simulink model "sliding_car"  (R2017a)
settings: Solver=VariableStepAuto  StartTime=0.0  StopTime=tf  RelTol=1e-3
values from neighbouring files (symbols this model uses):
  R = sys.descrip.syms(end-4)    [load_consts.m]
  sys = kinematic_model(sys)    [load_kin.m]
undefined symbols (not defined in the file or in its folder): a, Cp_1, Cp_2, Fz_1, Fz_2, g, Ic_33, Ii_11, Ii_21, Ii_22, Ii_31, Ii_32, Ii_33, Il_11, Il_21, Il_22, Il_31, Il_32, Il_33, Io_11, Io_21, Io_22, Io_31, Io_32, Io_33, Ir_11, Ir_21, Ir_22, Ir_31, Ir_32, Ir_33, L, Lc, mc, mi, ml, mo, mr, mu_1, mu_2, w, x0
(part 4 of 5)

== matlab function sliding_car/Vehicle/Steering automobile model/Auxiliary matrices/dC_1delta1 ==
  data: x input; qp input; kappa_1 input; kappa_2 input; alpha_1 input; alpha_2 input; dC_1delta output; dkappa_1 input; dkappa_2 input; dalpha_1 input; dalpha_2 input; w parameter; L parameter; R parameter
function dC_1delta = dKinematicMatrix(x, qp, kappa_1, kappa_2, alpha_1, alpha_2, ...
                                      dkappa_1, dkappa_2, dalpha_1, dalpha_2, ... 
                                      w, L, R)
% DCONSTRAINTMATRIX
%    A_1DELTA = DCONSTRAINTMATRIX(L,R,ALPHA_1,ALPHA_2,DELTA_I,DELTA_O,KAPPA_1,KAPPA_2,THETA,W)

%    This function was generated by the Symbolic Math Toolbox version 7.2.
%    16-Oct-2020 14:33:54
    
    x_pos =  x(1);
    y_pos =  x(2);
    theta =  x(3);

    delta_i = x(4);
    delta_o = x(5);

    phi_i = x(6);
    phi_l = x(7);
    phi_o = x(8);
    phi_r = x(9);
    
    p1 = x(10);
    p2 = x(11);
    p3 = x(12);
    
    xp = qp(1);
    yp = qp(2);
    thetap = qp(3);
    deltap_i = qp(4);
    deltap_o = qp(5);
    phip_i = qp(6);
    phip_o = qp(7);
    phip_r = qp(8);
    phip_l = qp(9);
    
    t2 = L.^2;
    t3 = tan(delta_i);
    t4 = t3.^2;
    t5 = tan(alpha_2);
    t6 = t3.*w;
    t7 = L+t6;
    t8 = 1.0./t7.^2;
    t9 = t2.*t4;
    t10 = w.^2;
    t11 = t4.*t10;
    t12 = L.*t3.*w.*2.0;
    t13 = t2+t9+t11+t12;
    t14 = t8.*t13;
    t15 = sqrt(t14);
    t16 = delta_i+theta;
    t17 = cos(t16);
    t18 = delta_o+theta;
    t19 = cos(t18);
    t20 = cos(delta_o);
    t21 = cos(delta_i);
    t22 = sin(delta_o);
    t23 = sin(delta_i);
    t24 = tan(alpha_1);
    t25 = sin(t16);
    t26 = 1.0./t7;
    t27 = L.*t3.*t26;
    t28 = atan(t27);
    t29 = t28+theta;
    t30 = cos(t29);
    t31 = sin(t29);
    t32 = t30.^2;
    t33 = t31.^2;
    t34 = sin(t18);
    t35 = kappa_2.*t2.*t5.*t15.*t19.*t23.*t30.*2.0;
    t36 = kappa_2.*t2.*t5.*t15.*t23.*t30.*t34.*2.0;
    t37 = kappa_2.*t2.*t5.*t15.*t23.*t31.*t34.*2.0;
    t38 = kappa_2.*t3.*t5.*t10.*t15.*t19.*t21.*t30;
    t39 = kappa_2.*t3.*t5.*t10.*t15.*t21.*t30.*t34;
    t40 = L.*kappa_2.*t5.*t15.*t19.*t21.*t30.*w;
    t41 = kappa_2.*t3.*t5.*t10.*t15.*t21.*t31.*t34;
    t42 = L.*kappa_2.*t5.*t15.*t21.*t30.*t34.*w;
    t43 = L.*kappa_2.*t5.*t15.*t21.*t31.*t34.*w;
    t44 = kappa_1.*kappa_2.*t2.*t5.*t15.*t19.*t21.*t24.*t31.*2.0;
    t45 = L.*kappa_2.*t3.*t5.*t15.*t19.*t23.*t30.*w.*2.0;
    t46 = L.*kappa_2.*t3.*t5.*t15.*t23.*t30.*t34.*w.*2.0;
    t47 = L.*kappa_2.*t3.*t5.*t15.*t23.*t31.*t34.*w.*2.0;
    t48 = kappa_1.*kappa_2.*t3.*t5.*t10.*t15.*t19.*t23.*t24.*t30;
    t49 = kappa_1.*kappa_2.*t3.*t5.*t10.*t15.*t23.*t24.*t30.*t34;
    t50 = L.*kappa_1.*kappa_2.*t5.*t15.*t19.*t23.*t24.*t30.*w;
    t51 = kappa_1.*kappa_2.*t3.*t5.*t10.*t15.*t23.*t24.*t31.*t34;
    t52 = L.*kappa_1.*kappa_2.*t5.*t15.*t23.*t24.*t30.*t34.*w;
    t53 = L.*kappa_1.*kappa_2.*t5.*t15.*t23.*t24.*t31.*t34.*w;
    t54 = L.*kappa_1.*kappa_2.*t3.*t5.*t15.*t19.*t21.*t24.*t31.*w.*2.0;
    t55 = t2.*t17.*t31.*2.0;
    t56 = t2.*t15.*t23.*t32.*2.0;
    t57 = t2.*t15.*t23.*t33.*2.0;
    t58 = t3.*t10.*t17.*t30;
    t59 = L.*t17.*t30.*w;
    t60 = t3.*t10.*t25.*t31;
    t61 = L.*t25.*t31.*w;
    t62 = t3.*t10.*t15.*t21.*t32;
    t63 = t3.*t10.*t15.*t21.*t33;
    t64 = L.*t15.*t21.*t32.*w;
    t65 = L.*t15.*t21.*t33.*w;
    t66 = L.*t3.*t17.*t31.*w.*3.0;
    t67 = kappa_1.*t2.*t17.*t24.*t30.*2.0;
    t68 = kappa_1.*t2.*t24.*t25.*t31.*2.0;
    t69 = L.*t3.*t15.*t23.*t32.*w.*2.0;
    t70 = L.*t3.*t15.*t23.*t33.*w.*2.0;
    t71 = kappa_2.*t3.*t5.*t10.*t17.*t19;
    t72 = L.*kappa_2.*t5.*t17.*t19.*w;
    t73 = kappa_2.*t3.*t5.*t10.*t25.*t34;
    t74 = kappa_1.*t2.*t3.*t17.*t24.*t31.*2.0;
    t75 = L.*kappa_2.*t5.*t25.*t34.*w;
    t76 = kappa_1.*t3.*t10.*t24.*t25.*t30;
    t77 = L.*kappa_1.*t24.*t25.*t30.*w;
    t78 = kappa_1.*t3.*t10.*t15.*t23.*t24.*t32;
    t79 = kappa_1.*t3.*t10.*t15.*t23.*t24.*t33;
    t80 = L.*kappa_1.*t15.*t23.*t24.*t32.*w;
    t81 = L.*kappa_1.*t3.*t17.*t24.*t30.*w.*3.0;
    t82 = L.*kappa_1.*t15.*t23.*t24.*t33.*w;
    t83 = kappa_2.*t2.*t5.*t15.*t17.*t20.*t30.*2.0;
    t84 = kappa_2.*t2.*t5.*t15.*t17.*t20.*t31.*2.0;
    t85 = L.*kappa_1.*t3.*t24.*t25.*t31.*w.*3.0;
    t86 = kappa_1.*kappa_2.*t2.*t5.*t17.*t24.*t34.*2.0;
    t87 = kappa_2.*t2.*t5.*t15.*t19.*t23.*t31.*2.0;
    t88 = kappa_2.*t2.*t5.*t15.*t20.*t25.*t31.*2.0;
    t89 = kappa_1.*kappa_2.*t2.*t3.*t5.*t17.*t24.*t34.*2.0;
    t90 = kappa_2.*t3.*t5.*t10.*t15.*t17.*t22.*t30;
    t91 = kappa_2.*t3.*t5.*t10.*t15.*t19.*t21.*t31;
    t92 = kappa_1.*kappa_2.*t3.*t5.*t10.*t19.*t24.*t25;
    t93 = kappa_2.*t3.*t5.*t10.*t15.*t17.*t22.*t31;
    t94 = L.*kappa_2.*t5.*t15.*t17.*t22.*t30.*w;
    t95 = L.*kappa_2.*t5.*t15.*t19.*t21.*t31.*w;
    t96 = kappa_2.*t3.*t5.*t10.*t15.*t22.*t25.*t31;
    t97 = L.*kappa_1.*kappa_2.*t5.*t19.*t24.*t25.*w;
    t98 = L.*kappa_2.*t5.*t15.*t17.*t22.*t31.*w;
    t99 = L.*kappa_2.*t5.*t15.*t22.*t25.*t31.*w;
    t100 = kappa_1.*kappa_2.*t2.*t5.*t15.*t20.*t24.*t25.*t30.*2.0;
    t101 = kappa_1.*kappa_2.*t2.*t5.*t15.*t21.*t24.*t30.*t34.*2.0;
    t102 = kappa_1.*kappa_2.*t2.*t5.*t15.*t20.*t24.*t25.*t31.*2.0;
    t103 = L.*kappa_2.*t3.*t5.*t15.*t17.*t20.*t30.*w.*2.0;
    t104 = L.*kappa_2.*t3.*t5.*t15.*t17.*t20.*t31.*w.*2.0;
    t105 = L.*kappa_1.*kappa_2.*t3.*t5.*t17.*t24.*t34.*w.*3.0;
    t106 = L.*kappa_2.*t3.*t5.*t15.*t19.*t23.*t31.*w.*2.0;
    t107 = L.*kappa_2.*t3.*t5.*t15.*t20.*t25.*t31.*w.*2.0;
    t108 = kappa_1.*kappa_2.*t2.*t5.*t15.*t17.*t20.*t24.*t30.*2.0;
    t109 = kappa_1.*kappa_2.*t3.*t5.*t10.*t15.*t17.*t22.*t24.*t30;
    t110 = kappa_1.*kappa_2.*t3.*t5.*t10.*t15.*t19.*t23.*t24.*t31;
    t111 = kappa_1.*kappa_2.*t3.*t5.*t10.*t15.*t22.*t24.*t25.*t30;
    t112 = L.*kappa_1.*kappa_2.*t5.*t15.*t17.*t22.*t24.*t30.*w;
    t113 = kappa_1.*kappa_2.*t3.*t5.*t10.*t15.*t22.*t24.*t25.*t31;
    t114 = L.*kappa_1.*kappa_2.*t5.*t15.*t19.*t23.*t24.*t31.*w;
    t115 = L.*kappa_1.*kappa_2.*t5.*t15.*t22.*t24.*t25.*t30.*w;
    t116 = L.*kappa_1.*kappa_2.*t5.*t15.*t22.*t24.*t25.*t31.*w;
    t117 = L.*kappa_1.*kappa_2.*t3.*t5.*t15.*t20.*t24.*t25.*t31.*w.*2.0;
    t118 = L.*kappa_1.*kappa_2.*t3.*t5.*t15.*t17.*t20.*t24.*t30.*w.*2.0;
    t119 = L.*kappa_1.*kappa_2.*t3.*t5.*t15.*t20.*t24.*t25.*t30.*w.*2.0;
    t120 = L.*kappa_1.*kappa_2.*t3.*t5.*t15.*t21.*t24.*t30.*t34.*w.*2.0;
    t121 = t5.^2;
    t122 = t121+1.0;
    t149 = t2.*t25.*t30.*2.0;
    t150 = t2.*t3.*t17.*t30.*2.0;
    t151 = t2.*t3.*t25.*t31.*2.0;
    t152 = L.*t3.*t25.*t30.*w.*3.0;
    t153 = kappa_2.*t2.*t5.*t17.*t19.*2.0;
    t154 = kappa_2.*t2.*t5.*t25.*t34.*2.0;
    t155 = kappa_2.*t2.*t3.*t5.*t17.*t19.*2.0;
    t156 = kappa_1.*t2.*t15.*t21.*t24.*t32.*2.0;
    t157 = kappa_2.*t2.*t3.*t5.*t25.*t34.*2.0;
    t158 = kappa_1.*t2.*t15.*t21.*t24.*t33.*2.0;
    t159 = kappa_1.*t2.*t3.*t24.*t25.*t30.*2.0;
    t160 = kappa_1.*t3.*t10.*t17.*t24.*t31;
    t161 = L.*kappa_1.*t17.*t24.*t31.*w;
    t162 = L.*kappa_2.*t3.*t5.*t17.*t19.*w.*3.0;
    t163 = L.*kappa_2.*t3.*t5.*t25.*t34.*w.*3.0;
    t164 = kappa_2.*t2.*t5.*t15.*t20.*t25.*t30.*2.0;
    t165 = kappa_1.*kappa_2.*t2.*t5.*t19.*t24.*t25.*2.0;
    t166 = L.*kappa_1.*t3.*t15.*t21.*t24.*t32.*w.*2.0;
    t167 = L.*kappa_1.*t3.*t15.*t21.*t24.*t33.*w.*2.0;
    t168 = kappa_1.*kappa_2.*t2.*t3.*t5.*t19.*t24.*t25.*2.0;
    t169 = kappa_1.*kappa_2.*t3.*t5.*t10.*t17.*t24.*t34;
    t170 = kappa_2.*t3.*t5.*t10.*t15.*t22.*t25.*t30;
    t171 = L.*kappa_1.*kappa_2.*t5.*t17.*t24.*t34.*w;
    t172 = L.*kappa_2.*t5.*t15.*t22.*t25.*t30.*w;
    t173 = kappa_1.*kappa_2.*t2.*t5.*t15.*t17.*t20.*t24.*t31.*2.0;
    t174 = kappa_1.*kappa_2.*t2.*t5.*t15.*t21.*t24.*t31.*t34.*2.0;
    t175 = L.*kappa_2.*t3.*t5.*t15.*t20.*t25.*t30.*w.*2.0;
    t176 = L.*kappa_1.*kappa_2.*t3.*t5.*t19.*t24.*t25.*w.*3.0;
    t177 = kappa_1.*kappa_2.*t2.*t5.*t15.*t19.*t21.*t24.*t30.*2.0;
    t178 = kappa_1.*kappa_2.*t3.*t5.*t10.*t15.*t17.*t22.*t24.*t31;
    t179 = L.*kappa_1.*kappa_2.*t5.*t15.*t17.*t22.*t24.*t31.*w;
    t180 = L.*kappa_1.*kappa_2.*t3.*t5.*t15.*t21.*t24.*t31.*t34.*w.*2.0;
    t181 = L.*kappa_1.*kappa_2.*t3.*t5.*t15.*t19.*t21.*t24.*t30.*w.*2.0;
    t182 = L.*kappa_1.*kappa_2.*t3.*t5.*t15.*t17.*t20.*t24.*t31.*w.*2.0;
    t123 = t35+t36+t37+t38+t39+t40+t41+t42+t43+t44+t45+t46+t47+t48+t49+t50+t51+t52+t53+t54+t55+t56+t57+t58+t59+t60+t61+t62+t63+t64+t65+t66+t67+t68+t69+t70+t71+t72+t73+t74+t75+t76+t77+t78+t79+t80+t81+t82+t83+t84+t85+t86-t87+t88+t89+t90-t91+t92+t93+t94-t95+t96+t97+t98+t99+t100-t101+t102+t103+t104+t105-t106+t107+t108+t109-t110+t111+t112+t113-t114+t115+t116+t117+t118+t119-t120-t149-t150-t151-t152-t153-t154-t155-t156-t157-t158-t159-t160-t161-t162-t163-t164-t165-t166-t167-t168-t169-t170-t171-t172-t173-t174-t175-t176-t177-t178-t179-t180-t181-t182;
    t124 = L.*R.*t17.*w;
    t125 = R.*t3.*t10.*t17;
    t126 = R.*t2.*t15.*t23.*t30.*2.0;
    t127 = R.*t3.*t10.*t15.*t21.*t30;
    t128 = L.*R.*t15.*t21.*t30.*w;
    t129 = R.*kappa_1.*t3.*t10.*t24.*t25;
    t130 = L.*R.*kappa_1.*t24.*t25.*w;
    t131 = L.*R.*t3.*t15.*t23.*t30.*w.*2.0;
    t132 = R.*kappa_2.*t2.*t5.*t15.*t17.*t20.*2.0;
    t133 = R.*kappa_2.*t2.*t5.*t15.*t23.*t34.*2.0;
    t134 = R.*kappa_2.*t3.*t5.*t10.*t15.*t17.*t22;
    t135 = R.*kappa_2.*t3.*t5.*t10.*t15.*t21.*t34;
    t136 = L.*R.*kappa_2.*t5.*t15.*t17.*t22.*w;
    t137 = L.*R.*kappa_2.*t5.*t15.*t21.*t34.*w;
    t138 = R.*kappa_1.*t3.*t10.*t15.*t23.*t24.*t30;
    t139 = L.*R.*kappa_1.*t15.*t23.*t24.*t30.*w;
    t140 = L.*R.*kappa_2.*t3.*t5.*t15.*t17.*t20.*w.*2.0;
    t141 = L.*R.*kappa_2.*t3.*t5.*t15.*t23.*t34.*w.*2.0;
    t142 = R.*kappa_1.*kappa_2.*t2.*t5.*t15.*t20.*t24.*t25.*2.0;
    t143 = R.*kappa_1.*kappa_2.*t3.*t5.*t10.*t15.*t22.*t24.*t25;
    t144 = R.*kappa_1.*kappa_2.*t3.*t5.*t10.*t15.*t23.*t24.*t34;
    t145 = L.*R.*kappa_1.*kappa_2.*t5.*t15.*t22.*t24.*t25.*w;
    t146 = L.*R.*kappa_1.*kappa_2.*t5.*t15.*t23.*t24.*t34.*w;
    t147 = L.*R.*kappa_1.*kappa_2.*t3.*t5.*t15.*t20.*t24.*t25.*w.*2.0;
    t185 = R.*t2.*t3.*t17.*2.0;
    t186 = R.*kappa_1.*t2.*t3.*t24.*t25.*2.0;
    t187 = R.*kappa_1.*t2.*t15.*t21.*t24.*t30.*2.0;
    t188 = L.*R.*kappa_1.*t3.*t15.*t21.*t24.*t30.*w.*2.0;
    t189 = R.*kappa_1.*kappa_2.*t2.*t5.*t15.*t21.*t24.*t34.*2.0;
    t190 = L.*R.*kappa_1.*kappa_2.*t3.*t5.*t15.*t21.*t24.*t34.*w.*2.0;
    t148 = t124+t125+t126+t127+t128+t129+t130+t131+t132+t133+t134+t135+t136+t137+t138+t139+t140+t141+t142+t143+t144+t145+t146+t147-t185-t186-t187-t188-t189-t190;
    t183 = 1.0./t123.^2;
    t184 = 1.0./t123;
    t191 = t4+1.0;
    t192 = t2.*t3.*t191.*2.0;
    t193 = t3.*t10.*t191.*2.0;
    t194 = L.*t191.*w.*2.0;
    t195 = t192+t193+t194;
    t196 = t8.*t195;
    t197 = 1.0./t7.^3;
    t200 = t13.*t191.*t197.*w.*2.0;
    t198 = t196-t200;
    t199 = 1.0./sqrt(t14);
    t201 = t2.*t4.*t8;
    t202 = t201+1.0;
    t203 = 1.0./t202;
    t204 = L.*t26.*t191;
    t206 = L.*t3.*t8.*t191.*w;
    t205 = t204-t206;
    t207 = kappa_2.*t2.*t5.*t17.*t34.*2.0;
    t208 = kappa_2.*t2.*t3.*t5.*t17.*t34.*2.0;
    t209 = kappa_2.*t3.*t5.*t10.*t19.*t25;
    t210 = L.*kappa_2.*t5.*t19.*t25.*w;
    t211 = L.*kappa_2.*t3.*t5.*t17.*t34.*w.*3.0;
    t212 = kappa_1.*kappa_2.*t2.*t5.*t17.*t19.*t24.*2.0;
    t213 = kappa_1.*kappa_2.*t2.*t5.*t24.*t25.*t34.*2.0;
    t214 = kappa_1.*kappa_2.*t2.*t3.*t5.*t17.*t19.*t24.*2.0;
    t215 = kappa_1.*kappa_2.*t2.*t3.*t5.*t24.*t25.*t34.*2.0;
    t216 = L.*kappa_1.*kappa_2.*t3.*t5.*t17.*t19.*t24.*w.*3.0;
    t217 = L.*kappa_1.*kappa_2.*t3.*t5.*t24.*t25.*t34.*w.*3.0;
    t218 = t24.^2;
    t219 = t218+1.0;
    t220 = R.*t2.*t3.*t25.*2.0;
    t221 = R.*kappa_1.*t3.*t10.*t17.*t24;
    t222 = L.*R.*kappa_1.*t17.*t24.*w;
    t223 = R.*kappa_2.*t2.*t5.*t15.*t19.*t23.*2.0;
    t224 = R.*kappa_2.*t3.*t5.*t10.*t15.*t19.*t21;
    t225 = L.*R.*kappa_2.*t5.*t15.*t19.*t21.*w;
    t226 = L.*R.*kappa_2.*t3.*t5.*t15.*t19.*t23.*w.*2.0;
    t227 = R.*kappa_1.*kappa_2.*t2.*t5.*t15.*t17.*t20.*t24.*2.0;
    t228 = R.*kappa_1.*kappa_2.*t3.*t5.*t10.*t15.*t17.*t22.*t24;
    t229 = R.*kappa_1.*kappa_2.*t3.*t5.*t10.*t15.*t19.*t23.*t24;
    t230 = L.*R.*kappa_1.*kappa_2.*t5.*t15.*t17.*t22.*t24.*w;
    t231 = L.*R.*kappa_1.*kappa_2.*t5.*t15.*t19.*t23.*t24.*w;
    t232 = L.*R.*kappa_1.*kappa_2.*t3.*t5.*t15.*t17.*t20.*t24.*w.*2.0;
    t233 = R.*kappa_1.*t2.*t15.*t21.*t24.*t31.*2.0;
    t234 = L.*R.*kappa_1.*t3.*t15.*t21.*t24.*t31.*w.*2.0;
    t235 = t3.*t5.*t10.*t17.*t19;
    t236 = L.*t5.*t17.*t19.*w;
    t237 = t3.*t5.*t10.*t25.*t34;
    t238 = L.*t5.*t25.*t34.*w;
    t239 = t2.*t5.*t15.*t17.*t20.*t30.*2.0;
    t240 = t2.*t5.*t15.*t17.*t20.*t31.*2.0;
    t241 = t2.*t5.*t15.*t19.*t23.*t30.*2.0;
    t242 = kappa_1.*t2.*t5.*t17.*t24.*t34.*2.0;
    t243 = t2.*t5.*t15.*t20.*t25.*t31.*2.0;
    t244 = t2.*t5.*t15.*t23.*t30.*t34.*2.0;
    t245 = t2.*t5.*t15.*t23.*t31.*t34.*2.0;
    t246 = kappa_1.*t2.*t3.*t5.*t17.*t24.*t34.*2.0;
    t247 = t3.*t5.*t10.*t15.*t19.*t21.*t30;
    t248 = t3.*t5.*t10.*t15.*t17.*t22.*t30;
    t249 = t3.*t5.*t10.*t15.*t21.*t30.*t34;
    t250 = L.*t5.*t15.*t19.*t21.*t30.*w;
    t251 = kappa_1.*t3.*t5.*t10.*t19.*t24.*t25;
    t252 = t3.*t5.*t10.*t15.*t17.*t22.*t31;
    t253 = t3.*t5.*t10.*t15.*t21.*t31.*t34;
    t254 = L.*t5.*t15.*t17.*t22.*t30.*w;
    t255 = L.*t5.*t15.*t21.*t30.*t34.*w;
    t256 = t3.*t5.*t10.*t15.*t22.*t25.*t31;
    t257 = L.*kappa_1.*t5.*t19.*t24.*t25.*w;
    t258 = L.*t5.*t15.*t17.*t22.*t31.*w;
    t259 = L.*t5.*t15.*t21.*t31.*t34.*w;
    t260 = L.*t5.*t15.*t22.*t25.*t31.*w;
    t261 = L.*t3.*t5.*t15.*t17.*t20.*t30.*w.*2.0;
    t262 = L.*t3.*t5.*t15.*t17.*t20.*t31.*w.*2.0;
    t263 = L.*t3.*t5.*t15.*t19.*t23.*t30.*w.*2.0;
    t264 = L.*kappa_1.*t3.*t5.*t17.*t24.*t34.*w.*3.0;
    t265 = L.*t3.*t5.*t15.*t20.*t25.*t31.*w.*2.0;
    t266 = L.*t3.*t5.*t15.*t23.*t30.*t34.*w.*2.0;
    t267 = L.*t3.*t5.*t15.*t23.*t31.*t34.*w.*2.0;
    t268 = kappa_1.*t2.*t5.*t15.*t17.*t20.*t24.*t30.*2.0;
    t269 = kappa_1.*t2.*t5.*t15.*t19.*t21.*t24.*t31.*2.0;
    t270 = kappa_1.*t2.*t5.*t15.*t20.*t24.*t25.*t30.*2.0;
    t271 = kappa_1.*t2.*t5.*t15.*t20.*t24.*t25.*t31.*2.0;
    t272 = kappa_1.*t3.*t5.*t10.*t15.*t17.*t22.*t24.*t30;
    t273 = kappa_1.*t3.*t5.*t10.*t15.*t19.*t23.*t24.*t30;
    t274 = kappa_1.*t3.*t5.*t10.*t15.*t22.*t24.*t25.*t30;
    t275 = kappa_1.*t3.*t5.*t10.*t15.*t23.*t24.*t30.*t34;
    t276 = L.*kappa_1.*t5.*t15.*t17.*t22.*t24.*t30.*w;
    t277 = L.*kappa_1.*t5.*t15.*t19.*t23.*t24.*t30.*w;
    t278 = kappa_1.*t3.*t5.*t10.*t15.*t22.*t24.*t25.*t31;
    t279 = kappa_1.*t3.*t5.*t10.*t15.*t23.*t24.*t31.*t34;
    t280 = L.*kappa_1.*t5.*t15.*t22.*t24.*t25.*t30.*w;
    t281 = L.*kappa_1.*t5.*t15.*t23.*t24.*t30.*t34.*w;
    t282 = L.*kappa_1.*t5.*t15.*t22.*t24.*t25.*t31.*w;
    t283 = L.*kappa_1.*t5.*t15.*t23.*t24.*t31.*t34.*w;
    t284 = L.*kappa_1.*t3.*t5.*t15.*t17.*t20.*t24.*t30.*w.*2.0;
    t285 = L.*kappa_1.*t3.*t5.*t15.*t19.*t21.*t24.*t31.*w.*2.0;
    t286 = L.*kappa_1.*t3.*t5.*t15.*t20.*t24.*t25.*t30.*w.*2.0;
    t287 = L.*kappa_1.*t3.*t5.*t15.*t20.*t24.*t25.*t31.*w.*2.0;
    t641 = t2.*t5.*t17.*t19.*2.0;
    t642 = t2.*t5.*t25.*t34.*2.0;
    t643 = t2.*t3.*t5.*t25.*t34.*2.0;
    t644 = t2.*t3.*t5.*t17.*t19.*2.0;
    t645 = L.*t3.*t5.*t17.*t19.*w.*3.0;
    t646 = L.*t3.*t5.*t25.*t34.*w.*3.0;
    t647 = t2.*t5.*t15.*t20.*t25.*t30.*2.0;
    t648 = kappa_1.*t2.*t5.*t19.*t24.*t25.*2.0;
    t649 = t2.*t5.*t15.*t19.*t23.*t31.*2.0;
    t650 = kappa_1.*t2.*t3.*t5.*t19.*t24.*t25.*2.0;
    t651 = t3.*t5.*t10.*t15.*t19.*t21.*t31;
    t652 = kappa_1.*t3.*t5.*t10.*t17.*t24.*t34;
    t653 = t3.*t5.*t10.*t15.*t22.*t25.*t30;
    t654 = L.*t5.*t15.*t19.*t21.*t31.*w;
    t655 = L.*kappa_1.*t5.*t17.*t24.*t34.*w;
    t656 = L.*t5.*t15.*t22.*t25.*t30.*w;
    t657 = L.*t3.*t5.*t15.*t20.*t25.*t30.*w.*2.0;
    t658 = L.*kappa_1.*t3.*t5.*t19.*t24.*t25.*w.*3.0;
    t659 = L.*t3.*t5.*t15.*t19.*t23.*t31.*w.*2.0;
    t660 = kappa_1.*t2.*t5.*t15.*t19.*t21.*t24.*t30.*2.0;
    t661 = kappa_1.*t2.*t5.*t15.*t17.*t20.*t24.*t31.*2.0;
    t662 = kappa_1.*t2.*t5.*t15.*t21.*t24.*t30.*t34.*2.0;
    t663 = kappa_1.*t2.*t5.*t15.*t21.*t24.*t31.*t34.*2.0;
    t664 = kappa_1.*t3.*t5.*t10.*t15.*t17.*t22.*t24.*t31;
    t665 = kappa_1.*t3.*t5.*t10.*t15.*t19.*t23.*t24.*t31;
    t666 = L.*kappa_1.*t5.*t15.*t17.*t22.*t24.*t31.*w;
    t667 = L.*kappa_1.*t5.*t15.*t19.*t23.*t24.*t31.*w;
    t668 = L.*kappa_1.*t3.*t5.*t15.*t19.*t21.*t24.*t30.*w.*2.0;
    t669 = L.*kappa_1.*t3.*t5.*t15.*t17.*t20.*t24.*t31.*w.*2.0;
    t670 = L.*kappa_1.*t3.*t5.*t15.*t21.*t24.*t30.*t34.*w.*2.0;
    t671 = L.*kappa_1.*t3.*t5.*t15.*t21.*t24.*t31.*t34.*w.*2.0;
    t288 = t235+t236+t237+t238+t239+t240+t241+t242+t243+t244+t245+t246+t247+t248+t249+t250+t251+t252+t253+t254+t255+t256+t257+t258+t259+t260+t261+t262+t263+t264+t265+t266+t267+t268+t269+t270+t271+t272+t273+t274+t275+t276+t277+t278+t279+t280+t281+t282+t283+t284+t285+t286+t287-t641-t642-t643-t644-t645-t646-t647-t648-t649-t650-t651-t652-t653-t654-t655-t656-t657-t658-t659-t660-t661-t662-t663-t664-t665-t666-t667-t668-t669-t670-t671;
    t290 = R.*t3.*t10.*t25;
    t291 = L.*R.*t25.*w;
    t292 = R.*t2.*t15.*t23.*t31.*2.0;
    t293 = R.*kappa_1.*t2.*t3.*t17.*t24.*2.0;
    t294 = R.*t3.*t10.*t15.*t21.*t31;
    t295 = L.*R.*t15.*t21.*t31.*w;
    t296 = L.*R.*t3.*t15.*t23.*t31.*w.*2.0;
    t297 = R.*kappa_2.*t2.*t5.*t15.*t20.*t25.*2.0;
    t298 = R.*kappa_2.*t3.*t5.*t10.*t15.*t22.*t25;
    t299 = L.*R.*kappa_2.*t5.*t15.*t22.*t25.*w;
    t300 = R.*kappa_1.*t3.*t10.*t15.*t23.*t24.*t31;
    t301 = L.*R.*kappa_1.*t15.*t23.*t24.*t31.*w;
    t302 = L.*R.*kappa_2.*t3.*t5.*t15.*t20.*t25.*w.*2.0;
    t303 = R.*kappa_1.*kappa_2.*t2.*t5.*t15.*t19.*t21.*t24.*2.0;
    t304 = L.*R.*kappa_1.*kappa_2.*t3.*t5.*t15.*t19.*t21.*t24.*w.*2.0;
    t289 = t220+t221+t222+t223+t224+t225+t226+t227+t228+t229+t230+t231+t232+t233+t234-t290-t291-t292-t293-t294-t295-t296-t297-t298-t299-t300-t301-t302-t303-t304;
    t305 = kappa_1.*t2.*t17.*t30.*t219.*2.0;
    t306 = kappa_1.*t2.*t25.*t31.*t219.*2.0;
    t307 = kappa_1.*t2.*t3.*t17.*t31.*t219.*2.0;
    t308 = kappa_1.*t3.*t10.*t25.*t30.*t219;
    t309 = L.*kappa_1.*t25.*t30.*t219.*w;
    t310 = kappa_1.*t3.*t10.*t15.*t23.*t32.*t219;
    t311 = kappa_1.*t3.*t10.*t15.*t23.*t33.*t219;
    t312 = L.*kappa_1.*t15.*t23.*t32.*t219.*w;
    t313 = L.*kappa_1.*t3.*t17.*t30.*t219.*w.*3.0;
    t314 = L.*kappa_1.*t15.*t23.*t33.*t219.*w;
    t315 = L.*kappa_1.*t3.*t25.*t31.*t219.*w.*3.0;
    t316 = kappa_1.*kappa_2.*t2.*t5.*t17.*t34.*t219.*2.0;
    t317 = kappa_1.*kappa_2.*t2.*t3.*t5.*t17.*t34.*t219.*2.0;
    t318 = kappa_1.*kappa_2.*t3.*t5.*t10.*t19.*t25.*t219;
    t319 = L.*kappa_1.*kappa_2.*t5.*t19.*t25.*t219.*w;
    t320 = L.*kappa_1.*kappa_2.*t3.*t5.*t17.*t34.*t219.*w.*3.0;
    t321 = kappa_1.*kappa_2.*t2.*t5.*t15.*t17.*t20.*t30.*t219.*2.0;
    t322 = kappa_1.*kappa_2.*t2.*t5.*t15.*t19.*t21.*t31.*t219.*2.0;
    t323 = kappa_1.*kappa_2.*t2.*t5.*t15.*t20.*t25.*t30.*t219.*2.0;
    t324 = kappa_1.*kappa_2.*t2.*t5.*t15.*t20.*t25.*t31.*t219.*2.0;
    t325 = kappa_1.*kappa_2.*t3.*t5.*t10.*t15.*t17.*t22.*t30.*t219;
    t326 = kappa_1.*kappa_2.*t3.*t5.*t10.*t15.*t19.*t23.*t30.*t219;
    t327 = kappa_1.*kappa_2.*t3.*t5.*t10.*t15.*t22.*t25.*t30.*t219;
    t328 = kappa_1.*kappa_2.*t3.*t5.*t10.*t15.*t23.*t30.*t34.*t219;
    t329 = L.*kappa_1.*kappa_2.*t5.*t15.*t17.*t22.*t30.*t219.*w;
    t330 = L.*kappa_1.*kappa_2.*t5.*t15.*t19.*t23.*t30.*t219.*w;
    t331 = kappa_1.*kappa_2.*t3.*t5.*t10.*t15.*t22.*t25.*t31.*t219;
    t332 = kappa_1.*kappa_2.*t3.*t5.*t10.*t15.*t23.*t31.*t34.*t219;
    t333 = L.*kappa_1.*kappa_2.*t5.*t15.*t22.*t25.*t30.*t219.*w;
    t334 = L.*kappa_1.*kappa_2.*t5.*t15.*t23.*t30.*t34.*t219.*w;
    t335 = L.*kappa_1.*kappa_2.*t5.*t15.*t22.*t25.*t31.*t219.*w;
    t336 = L.*kappa_1.*kappa_2.*t5.*t15.*t23.*t31.*t34.*t219.*w;
    t337 = L.*kappa_1.*kappa_2.*t3.*t5.*t15.*t17.*t20.*t30.*t219.*w.*2.0;
    t338 = L.*kappa_1.*kappa_2.*t3.*t5.*t15.*t19.*t21.*t31.*t219.*w.*2.0;
    t339 = L.*kappa_1.*kappa_2.*t3.*t5.*t15.*t20.*t25.*t30.*t219.*w.*2.0;
    t340 = L.*kappa_1.*kappa_2.*t3.*t5.*t15.*t20.*t25.*t31.*t219.*w.*2.0;
    t731 = kappa_1.*t2.*t15.*t21.*t32.*t219.*2.0;
    t732 = kappa_1.*t2.*t15.*t21.*t33.*t219.*2.0;
    t733 = kappa_1.*t2.*t3.*t25.*t30.*t219.*2.0;
    t734 = kappa_1.*t3.*t10.*t17.*t31.*t219;
    t735 = L.*kappa_1.*t17.*t31.*t219.*w;
    t736 = kappa_1.*kappa_2.*t2.*t5.*t19.*t25.*t219.*2.0;
    t737 = L.*kappa_1.*t3.*t15.*t21.*t32.*t219.*w.*2.0;
    t738 = L.*kappa_1.*t3.*t15.*t21.*t33.*t219.*w.*2.0;
    t739 = kappa_1.*kappa_2.*t2.*t3.*t5.*t19.*t25.*t219.*2.0;
    t740 = kappa_1.*kappa_2.*t3.*t5.*t10.*t17.*t34.*t219;
    t741 = L.*kappa_1.*kappa_2.*t5.*t17.*t34.*t219.*w;
    t742 = L.*kappa_1.*kappa_2.*t3.*t5.*t19.*t25.*t219.*w.*3.0;
    t743 = kappa_1.*kappa_2.*t2.*t5.*t15.*t19.*t21.*t30.*t219.*2.0;
    t744 = kappa_1.*kappa_2.*t2.*t5.*t15.*t17.*t20.*t31.*t219.*2.0;
    t745 = kappa_1.*kappa_2.*t2.*t5.*t15.*t21.*t30.*t34.*t219.*2.0;
    t746 = kappa_1.*kappa_2.*t2.*t5.*t15.*t21.*t31.*t34.*t219.*2.0;
    t747 = kappa_1.*kappa_2.*t3.*t5.*t10.*t15.*t17.*t22.*t31.*t219;
    t748 = kappa_1.*kappa_2.*t3.*t5.*t10.*t15.*t19.*t23.*t31.*t219;
    t749 = L.*kappa_1.*kappa_2.*t5.*t15.*t17.*t22.*t31.*t219.*w;
    t750 = L.*kappa_1.*kappa_2.*t5.*t15.*t19.*t23.*t31.*t219.*w;
    t751 = L.*kappa_1.*kappa_2.*t3.*t5.*t15.*t19.*t21.*t30.*t219.*w.*2.0;
    t752 = L.*kappa_1.*kappa_2.*t3.*t5.*t15.*t17.*t20.*t31.*t219.*w.*2.0;
    t753 = L.*kappa_1.*kappa_2.*t3.*t5.*t15.*t21.*t30.*t34.*t219.*w.*2.0;
    t754 = L.*kappa_1.*kappa_2.*t3.*t5.*t15.*t21.*t31.*t34.*t219.*w.*2.0;
    t341 = t305+t306+t307+t308+t309+t310+t311+t312+t313+t314+t315+t316+t317+t318+t319+t320+t321+t322+t323+t324+t325+t326+t327+t328+t329+t330+t331+t332+t333+t334+t335+t336+t337+t338+t339+t340-t731-t732-t733-t734-t735-t736-t737-t738-t739-t740-t741-t742-t743-t744-t745-t746-t747-t748-t749-t750-t751-t752-t753-t754;
    t342 = kappa_2.*t2.*t5.*t19.*t25.*2.0;
    t343 = kappa_2.*t2.*t3.*t5.*t19.*t25.*2.0;
    t344 = kappa_2.*t3.*t5.*t10.*t17.*t34;
    t345 = L.*kappa_2.*t5.*t17.*t34.*w;
    t346 = L.*kappa_2.*t3.*t5.*t19.*t25.*w.*3.0;
    t347 = kappa_2.*t2.*t5.*t15.*t22.*t25.*t30.*2.0;
    t348 = kappa_2.*t3.*t5.*t10.*t15.*t17.*t20.*t30;
    t349 = kappa_1.*kappa_2.*t3.*t5.*t10.*t17.*t19.*t24;
    t350 = kappa_2.*t3.*t5.*t10.*t15.*t17.*t20.*t31;
    t351 = L.*kappa_2.*t5.*t15.*t17.*t20.*t30.*w;
    t352 = kappa_2.*t3.*t5.*t10.*t15.*t20.*t25.*t31;
    t353 = L.*kappa_1.*kappa_2.*t5.*t17.*t19.*t24.*w;
    t354 = L.*kappa_2.*t5.*t15.*t17.*t20.*t31.*w;
    t355 = kappa_1.*kappa_2.*t3.*t5.*t10.*t24.*t25.*t34;
    t356 = L.*kappa_2.*t5.*t15.*t20.*t25.*t31.*w;
    t357 = L.*kappa_1.*kappa_2.*t5.*t24.*t25.*t34.*w;
    t358 = kappa_1.*kappa_2.*t2.*t5.*t15.*t17.*t22.*t24.*t31.*2.0;
    t359 = L.*kappa_2.*t3.*t5.*t15.*t22.*t25.*t30.*w.*2.0;
    t360 = kappa_1.*kappa_2.*t3.*t5.*t10.*t15.*t20.*t24.*t25.*t30;
    t361 = L.*kappa_1.*kappa_2.*t5.*t15.*t17.*t20.*t24.*t30.*w;
    t362 = kappa_1.*kappa_2.*t3.*t5.*t10.*t15.*t20.*t24.*t25.*t31;
    t363 = L.*kappa_1.*kappa_2.*t5.*t15.*t20.*t24.*t25.*t30.*w;
    t364 = L.*kappa_1.*kappa_2.*t5.*t15.*t20.*t24.*t25.*t31.*w;
    t365 = kappa_1.*kappa_2.*t3.*t5.*t10.*t15.*t17.*t20.*t24.*t30;
    t366 = L.*kappa_1.*kappa_2.*t3.*t5.*t15.*t17.*t22.*t24.*t31.*w.*2.0;
    t367 = kappa_2.*t3.*t10.*t17.*t19.*t122;
    t368 = L.*kappa_2.*t17.*t19.*t122.*w;
    t369 = kappa_2.*t3.*t10.*t25.*t34.*t122;
    t370 = L.*kappa_2.*t25.*t34.*t122.*w;
    t371 = kappa_2.*t2.*t15.*t17.*t20.*t30.*t122.*2.0;
    t372 = kappa_2.*t2.*t15.*t17.*t20.*t31.*t122.*2.0;
    t373 = kappa_2.*t2.*t15.*t19.*t23.*t30.*t122.*2.0;
    t374 = kappa_1.*kappa_2.*t2.*t17.*t24.*t34.*t122.*2.0;
    t375 = kappa_2.*t2.*t15.*t20.*t25.*t31.*t122.*2.0;
    t376 = kappa_2.*t2.*t15.*t23.*t30.*t34.*t122.*2.0;
    t377 = kappa_2.*t2.*t15.*t23.*t31.*t34.*t122.*2.0;
    t378 = kappa_1.*kappa_2.*t2.*t3.*t17.*t24.*t34.*t122.*2.0;
    t379 = kappa_2.*t3.*t10.*t15.*t19.*t21.*t30.*t122;
    t380 = kappa_2.*t3.*t10.*t15.*t17.*t22.*t30.*t122;
    t381 = kappa_2.*t3.*t10.*t15.*t21.*t30.*t34.*t122;
    t382 = L.*kappa_2.*t15.*t19.*t21.*t30.*t122.*w;
    t383 = kappa_1.*kappa_2.*t3.*t10.*t19.*t24.*t25.*t122;
    t384 = kappa_2.*t3.*t10.*t15.*t17.*t22.*t31.*t122;
    t385 = kappa_2.*t3.*t10.*t15.*t21.*t31.*t34.*t122;
    t386 = L.*kappa_2.*t15.*t17.*t22.*t30.*t122.*w;
    t387 = L.*kappa_2.*t15.*t21.*t30.*t34.*t122.*w;
    t388 = kappa_2.*t3.*t10.*t15.*t22.*t25.*t31.*t122;
    t389 = L.*kappa_1.*kappa_2.*t19.*t24.*t25.*t122.*w;
    t390 = L.*kappa_2.*t15.*t17.*t22.*t31.*t122.*w;
    t391 = L.*kappa_2.*t15.*t21.*t31.*t34.*t122.*w;
    t392 = L.*kappa_2.*t15.*t22.*t25.*t31.*t122.*w;
    t393 = L.*kappa_2.*t3.*t15.*t17.*t20.*t30.*t122.*w.*2.0;
    t394 = L.*kappa_2.*t3.*t15.*t17.*t20.*t31.*t122.*w.*2.0;
    t395 = L.*kappa_2.*t3.*t15.*t19.*t23.*t30.*t122.*w.*2.0;
    t396 = L.*kappa_1.*kappa_2.*t3.*t17.*t24.*t34.*t122.*w.*3.0;
    t397 = L.*kappa_2.*t3.*t15.*t20.*t25.*t31.*t122.*w.*2.0;
    t398 = L.*kappa_2.*t3.*t15.*t23.*t30.*t34.*t122.*w.*2.0;
    t399 = L.*kappa_2.*t3.*t15.*t23.*t31.*t34.*t122.*w.*2.0;
    t400 = kappa_1.*kappa_2.*t2.*t15.*t17.*t20.*t24.*t30.*t122.*2.0;
    t401 = kappa_1.*kappa_2.*t2.*t15.*t19.*t21.*t24.*t31.*t122.*2.0;
    t402 = kappa_1.*kappa_2.*t2.*t15.*t20.*t24.*t25.*t30.*t122.*2.0;
    t403 = kappa_1.*kappa_2.*t2.*t15.*t20.*t24.*t25.*t31.*t122.*2.0;
    t404 = kappa_1.*kappa_2.*t3.*t10.*t15.*t17.*t22.*t24.*t30.*t122;
    t405 = kappa_1.*kappa_2.*t3.*t10.*t15.*t19.*t23.*t24.*t30.*t122;
    t406 = kappa_1.*kappa_2.*t3.*t10.*t15.*t22.*t24.*t25.*t30.*t122;
    t407 = kappa_1.*kappa_2.*t3.*t10.*t15.*t23.*t24.*t30.*t34.*t122;
    t408 = L.*kappa_1.*kappa_2.*t15.*t17.*t22.*t24.*t30.*t122.*w;
    t409 = L.*kappa_1.*kappa_2.*t15.*t19.*t23.*t24.*t30.*t122.*w;
    t410 = kappa_1.*kappa_2.*t3.*t10.*t15.*t22.*t24.*t25.*t31.*t122;
    t411 = kappa_1.*kappa_2.*t3.*t10.*t15.*t23.*t24.*t31.*t34.*t122;
    t412 = L.*kappa_1.*kappa_2.*t15.*t22.*t24.*t25.*t30.*t122.*w;
    t413 = L.*kappa_1.*kappa_2.*t15.*t23.*t24.*t30.*t34.*t122.*w;
    t414 = L.*kappa_1.*kappa_2.*t15.*t22.*t24.*t25.*t31.*t122.*w;
    t415 = L.*kappa_1.*kappa_2.*t15.*t23.*t24.*t31.*t34.*t122.*w;
    t416 = L.*kappa_1.*kappa_2.*t3.*t15.*t17.*t20.*t24.*t30.*t122.*w.*2.0;
    t417 = L.*kappa_1.*kappa_2.*t3.*t15.*t19.*t21.*t24.*t31.*t122.*w.*2.0;
    t418 = L.*kappa_1.*kappa_2.*t3.*t15.*t20.*t24.*t25.*t30.*t122.*w.*2.0;
    t419 = L.*kappa_1.*kappa_2.*t3.*t15.*t20.*t24.*t25.*t31.*t122.*w.*2.0;
    t700 = kappa_2.*t2.*t17.*t19.*t122.*2.0;
    t701 = kappa_2.*t2.*t25.*t34.*t122.*2.0;
    t702 = kappa_2.*t2.*t3.*t17.*t19.*t122.*2.0;
    t703 = kappa_2.*t2.*t3.*t25.*t34.*t122.*2.0;
    t704 = L.*kappa_2.*t3.*t17.*t19.*t122.*w.*3.0;
    t705 = L.*kappa_2.*t3.*t25.*t34.*t122.*w.*3.0;
    t706 = kappa_2.*t2.*t15.*t20.*t25.*t30.*t122.*2.0;
    t707 = kappa_1.*kappa_2.*t2.*t19.*t24.*t25.*t122.*2.0;
    t708 = kappa_2.*t2.*t15.*t19.*t23.*t31.*t122.*2.0;
    t709 = kappa_1.*kappa_2.*t2.*t3.*t19.*t24.*t25.*t122.*2.0;
    t710 = kappa_2.*t3.*t10.*t15.*t19.*t21.*t31.*t122;
    t711 = kappa_1.*kappa_2.*t3.*t10.*t17.*t24.*t34.*t122;
    t712 = kappa_2.*t3.*t10.*t15.*t22.*t25.*t30.*t122;
    t713 = L.*kappa_2.*t15.*t19.*t21.*t31.*t122.*w;
    t714 = L.*kappa_1.*kappa_2.*t17.*t24.*t34.*t122.*w;
    t715 = L.*kappa_2.*t15.*t22.*t25.*t30.*t122.*w;
    t716 = L.*kappa_2.*t3.*t15.*t20.*t25.*t30.*t122.*w.*2.0;
    t717 = L.*kappa_1.*kappa_2.*t3.*t19.*t24.*t25.*t122.*w.*3.0;
    t718 = L.*kappa_2.*t3.*t15.*t19.*t23.*t31.*t122.*w.*2.0;
    t719 = kappa_1.*kappa_2.*t2.*t15.*t19.*t21.*t24.*t30.*t122.*2.0;
    t720 = kappa_1.*kappa_2.*t2.*t15.*t17.*t20.*t24.*t31.*t122.*2.0;
    t721 = kappa_1.*kappa_2.*t2.*t15.*t21.*t24.*t30.*t34.*t122.*2.0;
    t722 = kappa_1.*kappa_2.*t2.*t15.*t21.*t24.*t31.*t34.*t122.*2.0;
    t723 = kappa_1.*kappa_2.*t3.*t10.*t15.*t17.*t22.*t24.*t31.*t122;
    t724 = kappa_1.*kappa_2.*t3.*t10.*t15.*t19.*t23.*t24.*t31.*t122;
    t725 = L.*kappa_1.*kappa_2.*t15.*t17.*t22.*t24.*t31.*t122.*w;
    t726 = L.*kappa_1.*kappa_2.*t15.*t19.*t23.*t24.*t31.*t122.*w;
    t727 = L.*kappa_1.*kappa_2.*t3.*t15.*t19.*t21.*t24.*t30.*t122.*w.*2.0;
    t728 = L.*kappa_1.*kappa_2.*t3.*t15.*t17.*t20.*t24.*t31.*t122.*w.*2.0;
    t729 = L.*kappa_1.*kappa_2.*t3.*t15.*t21.*t24.*t30.*t34.*t122.*w.*2.0;
    t730 = L.*kappa_1.*kappa_2.*t3.*t15.*t21.*t24.*t31.*t34.*t122.*w.*2.0;
    t420 = t367+t368+t369+t370+t371+t372+t373+t374+t375+t376+t377+t378+t379+t380+t381+t382+t383+t384+t385+t386+t387+t388+t389+t390+t391+t392+t393+t394+t395+t396+t397+t398+t399+t400+t401+t402+t403+t404+t405+t406+t407+t408+t409+t410+t411+t412+t413+t414+t415+t416+t417+t418+t419-t700-t701-t702-t703-t704-t705-t706-t707-t708-t709-t710-t711-t712-t713-t714-t715-t716-t717-t718-t719-t720-t721-t722-t723-t724-t725-t726-t727-t728-t729-t730;
    t421 = t2.*t17.*t24.*t30.*2.0;
    t422 = t2.*t24.*t25.*t31.*2.0;
    t423 = t2.*t3.*t17.*t24.*t31.*2.0;
    t424 = t3.*t10.*t24.*t25.*t30;
    t425 = L.*t24.*t25.*t30.*w;
    t426 = t3.*t10.*t15.*t23.*t24.*t32;
    t427 = t3.*t10.*t15.*t23.*t24.*t33;
    t428 = L.*t15.*t23.*t24.*t32.*w;
    t429 = L.*t3.*t17.*t24.*t30.*w.*3.0;
    t430 = L.*t15.*t23.*t24.*t33.*w;
    t431 = L.*t3.*t24.*t25.*t31.*w.*3.0;
    t432 = kappa_2.*t2.*t5.*t17.*t24.*t34.*2.0;
    t433 = kappa_2.*t2.*t3.*t5.*t17.*t24.*t34.*2.0;
    t434 = kappa_2.*t3.*t5.*t10.*t19.*t24.*t25;
    t435 = L.*kappa_2.*t5.*t19.*t24.*t25.*w;
    t436 = L.*kappa_2.*t3.*t5.*t17.*t24.*t34.*w.*3.0;
    t437 = kappa_2.*t2.*t5.*t15.*t17.*t20.*t24.*t30.*2.0;
    t438 = kappa_2.*t2.*t5.*t15.*t19.*t21.*t24.*t31.*2.0;
    t439 = kappa_2.*t2.*t5.*t15.*t20.*t24.*t25.*t30.*2.0;
    t440 = kappa_2.*t2.*t5.*t15.*t20.*t24.*t25.*t31.*2.0;
    t441 = kappa_2.*t3.*t5.*t10.*t15.*t17.*t22.*t24.*t30;
    t442 = kappa_2.*t3.*t5.*t10.*t15.*t19.*t23.*t24.*t30;
    t443 = kappa_2.*t3.*t5.*t10.*t15.*t22.*t24.*t25.*t30;
    t444 = kappa_2.*t3.*t5.*t10.*t15.*t23.*t24.*t30.*t34;
    t445 = L.*kappa_2.*t5.*t15.*t17.*t22.*t24.*t30.*w;
    t446 = L.*kappa_2.*t5.*t15.*t19.*t23.*t24.*t30.*w;
    t447 = kappa_2.*t3.*t5.*t10.*t15.*t22.*t24.*t25.*t31;
    t448 = kappa_2.*t3.*t5.*t10.*t15.*t23.*t24.*t31.*t34;
    t449 = L.*kappa_2.*t5.*t15.*t22.*t24.*t25.*t30.*w;
    t450 = L.*kappa_2.*t5.*t15.*t23.*t24.*t30.*t34.*w;
    t451 = L.*kappa_2.*t5.*t15.*t22.*t24.*t25.*t31.*w;
    t452 = L.*kappa_2.*t5.*t15.*t23.*t24.*t31.*t34.*w;
    t453 = L.*kappa_2.*t3.*t5.*t15.*t17.*t20.*t24.*t30.*w.*2.0;
    t454 = L.*kappa_2.*t3.*t5.*t15.*t19.*t21.*t24.*t31.*w.*2.0;
    t455 = L.*kappa_2.*t3.*t5.*t15.*t20.*t24.*t25.*t30.*w.*2.0;
    t456 = L.*kappa_2.*t3.*t5.*t15.*t20.*t24.*t25.*t31.*w.*2.0;
    t676 = t2.*t15.*t21.*t24.*t32.*2.0;
    t677 = t2.*t15.*t21.*t24.*t33.*2.0;
    t678 = t2.*t3.*t24.*t25.*t30.*2.0;
    t679 = t3.*t10.*t17.*t24.*t31;
    t680 = L.*t17.*t24.*t31.*w;
    t681 = kappa_2.*t2.*t5.*t19.*t24.*t25.*2.0;
    t682 = L.*t3.*t15.*t21.*t24.*t33.*w.*2.0;
    t683 = kappa_2.*t2.*t3.*t5.*t19.*t24.*t25.*2.0;
    t684 = kappa_2.*t3.*t5.*t10.*t17.*t24.*t34;
    t685 = L.*kappa_2.*t5.*t17.*t24.*t34.*w;
    t686 = L.*t3.*t15.*t21.*t24.*t32.*w.*2.0;
    t687 = L.*kappa_2.*t3.*t5.*t19.*t24.*t25.*w.*3.0;
    t688 = kappa_2.*t2.*t5.*t15.*t19.*t21.*t24.*t30.*2.0;
    t689 = kappa_2.*t2.*t5.*t15.*t17.*t20.*t24.*t31.*2.0;
    t690 = kappa_2.*t2.*t5.*t15.*t21.*t24.*t30.*t34.*2.0;
    t691 = kappa_2.*t2.*t5.*t15.*t21.*t24.*t31.*t34.*2.0;
    t692 = kappa_2.*t3.*t5.*t10.*t15.*t17.*t22.*t24.*t31;
    t693 = kappa_2.*t3.*t5.*t10.*t15.*t19.*t23.*t24.*t31;
    t694 = L.*kappa_2.*t5.*t15.*t17.*t22.*t24.*t31.*w;
    t695 = L.*kappa_2.*t5.*t15.*t19.*t23.*t24.*t31.*w;
    t696 = L.*kappa_2.*t3.*t5.*t15.*t19.*t21.*t24.*t30.*w.*2.0;
    t697 = L.*kappa_2.*t3.*t5.*t15.*t17.*t20.*t24.*t31.*w.*2.0;
    t698 = L.*kappa_2.*t3.*t5.*t15.*t21.*t24.*t30.*t34.*w.*2.0;
    t699 = L.*kappa_2.*t3.*t5.*t15.*t21.*t24.*t31.*t34.*w.*2.0;
    t457 = t421+t422+t423+t424+t425+t426+t427+t428+t429+t430+t431+...
           t432+t433+t434+t435+t436+t437+t438+t439+t440+t441+t442+...
           t443+t444+t445+t446+t447+t448+t449+t450+t451+t452+t453+t454+...
           t455+t456-t676-t677-t678-t679-t680-t681-t682-t683-t684-t685-...
           t686-t687-t688-t689-t690-t691-t692-t693-t694-t695-t696-t697-t698-t699;
    t458 = t2.*t15.*t21.*t32.*2.0;
    t459 = t10.*t17.*t30.*t191;
    t460 = t2.*t15.*t21.*t33.*2.0;
    t461 = t10.*t25.*t31.*t191;
    t462 = t2.*t3.*t25.*t30.*2.0;
    t463 = t3.*t10.*t17.*t31;
    t464 = L.*t17.*t31.*w;
    t465 = t2.*t25.*t31.*t203.*t205.*2.0;
    t466 = t10.*t15.*t21.*t33.*t191;
    t467 = L.*t17.*t31.*t191.*w.*3.0;
    t468 = kappa_1.*t2.*t17.*t24.*t31.*2.0;
    t469 = t2.*t23.*t32.*t198.*t199;
    t470 = t2.*t17.*t30.*t203.*t205.*2.0;
    t471 = t2.*t23.*t33.*t198.*t199;
    t472 = t10.*t15.*t21.*t32.*t191;
    t473 = L.*t15.*t23.*t33.*t191.*w.*2.0;
    t474 = L.*t25.*t30.*t203.*t205.*w;
    t475 = L.*t3.*t15.*t21.*t32.*w.*2.0;
    t476 = L.*t3.*t15.*t21.*t33.*w.*2.0;
    t477 = kappa_2.*t5.*t10.*t17.*t19.*t191;
    t478 = kappa_2.*t5.*t10.*t25.*t34.*t191;
    t479 = kappa_1.*t2.*t17.*t24.*t31.*t191.*2.0;
    t480 = kappa_1.*t2.*t15.*t23.*t24.*t32.*2.0;
    t481 = kappa_1.*t10.*t24.*t25.*t30.*t191;
    t482 = kappa_1.*t2.*t15.*t23.*t24.*t33.*2.0;
    t483 = kappa_1.*t3.*t10.*t17.*t24.*t30;
    t484 = t2.*t3.*t17.*t31.*t203.*t205.*2.0;
    t485 = t3.*t10.*t21.*t32.*t198.*t199.*(1.0./2.0);
    t486 = L.*kappa_1.*t17.*t24.*t30.*w;
    t487 = t3.*t10.*t21.*t33.*t198.*t199.*(1.0./2.0);
    t488 = kappa_1.*t3.*t10.*t24.*t25.*t31;
    t489 = L.*t21.*t32.*t198.*t199.*w.*(1.0./2.0);
    t490 = L.*t21.*t33.*t198.*t199.*w.*(1.0./2.0);
    t491 = L.*kappa_1.*t24.*t25.*t31.*w;
    t492 = t3.*t10.*t25.*t30.*t203.*t205;
    t493 = L.*t15.*t23.*t32.*t191.*w.*2.0;
    t494 = kappa_1.*t2.*t24.*t25.*t30.*t203.*t205.*2.0;
    t495 = kappa_1.*t10.*t15.*t23.*t24.*t32.*t191;
    t496 = kappa_1.*t10.*t15.*t23.*t24.*t33.*t191;
    t497 = L.*kappa_1.*t17.*t24.*t30.*t191.*w.*3.0;
    t498 = kappa_1.*t3.*t10.*t15.*t21.*t24.*t32;
    t499 = L.*kappa_1.*t24.*t25.*t31.*t191.*w.*3.0;
    t500 = kappa_1.*t3.*t10.*t15.*t21.*t24.*t33;
    t501 = L.*kappa_1.*t15.*t21.*t24.*t32.*w;
    t502 = L.*kappa_1.*t15.*t21.*t24.*t33.*w;
    t503 = kappa_2.*t2.*t5.*t15.*t19.*t21.*t30.*2.0;
    t504 = L.*kappa_1.*t3.*t17.*t24.*t31.*w.*3.0;
    t505 = kappa_2.*t2.*t5.*t15.*t21.*t30.*t34.*2.0;
    t506 = L.*t3.*t23.*t32.*t198.*t199.*w;
    t507 = L.*t3.*t17.*t30.*t203.*t205.*w.*3.0;
    t508 = kappa_2.*t2.*t5.*t15.*t21.*t31.*t34.*2.0;
    t509 = L.*t3.*t23.*t33.*t198.*t199.*w;
    t510 = L.*t3.*t25.*t31.*t203.*t205.*w.*3.0;
    t511 = kappa_1.*t2.*t3.*t24.*t25.*t31.*t203.*t205.*2.0;
    t512 = kappa_1.*t3.*t10.*t23.*t24.*t32.*t198.*t199.*(1.0./2.0);
    t513 = kappa_1.*t3.*t10.*t23.*t24.*t33.*t198.*t199.*(1.0./2.0);
    t514 = L.*kappa_1.*t23.*t24.*t32.*t198.*t199.*w.*(1.0./2.0);
    t515 = L.*kappa_1.*t23.*t24.*t33.*t198.*t199.*w.*(1.0./2.0);
    t516 = kappa_2.*t2.*t5.*t17.*t20.*t30.*t198.*t199;
    t517 = kappa_2.*t2.*t5.*t17.*t20.*t31.*t198.*t199;
    t518 = kappa_2.*t2.*t5.*t19.*t23.*t30.*t198.*t199;
    t519 = kappa_2.*t2.*t5.*t20.*t25.*t31.*t198.*t199;
    t520 = kappa_2.*t2.*t5.*t23.*t30.*t34.*t198.*t199;
    t521 = kappa_1.*kappa_2.*t2.*t5.*t17.*t24.*t34.*t191.*2.0;
    t522 = kappa_2.*t5.*t10.*t15.*t19.*t21.*t30.*t191;
    t523 = kappa_2.*t2.*t5.*t23.*t31.*t34.*t198.*t199;
    t524 = L.*kappa_1.*t3.*t15.*t23.*t24.*t32.*w.*2.0;
    t525 = kappa_2.*t5.*t10.*t15.*t17.*t22.*t30.*t191;
    t526 = kappa_2.*t5.*t10.*t15.*t21.*t30.*t34.*t191;
    t527 = L.*kappa_1.*t3.*t15.*t23.*t24.*t33.*w.*2.0;
    t528 = kappa_1.*kappa_2.*t5.*t10.*t19.*t24.*t25.*t191;
    t529 = kappa_2.*t5.*t10.*t15.*t17.*t22.*t31.*t191;
    t530 = kappa_2.*t5.*t10.*t15.*t21.*t31.*t34.*t191;
    t531 = kappa_2.*t5.*t10.*t15.*t22.*t25.*t31.*t191;
    t532 = kappa_2.*t3.*t5.*t10.*t15.*t19.*t23.*t31;
    t533 = L.*kappa_2.*t5.*t15.*t19.*t23.*t31.*w;
    t534 = kappa_1.*t2.*t3.*t17.*t24.*t30.*t203.*t205.*2.0;
    t535 = kappa_1.*kappa_2.*t2.*t5.*t15.*t19.*t23.*t24.*t30.*2.0;
    t536 = kappa_1.*kappa_2.*t2.*t5.*t15.*t23.*t24.*t30.*t34.*2.0;
    t537 = kappa_2.*t2.*t5.*t15.*t17.*t20.*t30.*t203.*t205.*2.0;
    t538 = L.*kappa_1.*t3.*t24.*t25.*t30.*t203.*t205.*w.*3.0;
    t539 = kappa_1.*kappa_2.*t2.*t5.*t15.*t23.*t24.*t31.*t34.*2.0;
    t540 = kappa_2.*t2.*t5.*t15.*t20.*t25.*t30.*t203.*t205.*2.0;
    t541 = kappa_2.*t2.*t5.*t15.*t20.*t25.*t31.*t203.*t205.*2.0;
    t542 = kappa_2.*t2.*t5.*t15.*t23.*t30.*t34.*t203.*t205.*2.0;
    t543 = kappa_2.*t3.*t5.*t10.*t19.*t21.*t30.*t198.*t199.*(1.0./2.0);
    t544 = kappa_2.*t3.*t5.*t10.*t17.*t22.*t30.*t198.*t199.*(1.0./2.0);
    t545 = kappa_2.*t3.*t5.*t10.*t21.*t30.*t34.*t198.*t199.*(1.0./2.0);
    t546 = L.*kappa_2.*t5.*t19.*t21.*t30.*t198.*t199.*w.*(1.0./2.0);
    t547 = L.*kappa_2.*t5.*t15.*t17.*t20.*t30.*t191.*w.*2.0;
    t548 = kappa_2.*t3.*t5.*t10.*t17.*t22.*t31.*t198.*t199.*(1.0./2.0);
    t549 = kappa_2.*t3.*t5.*t10.*t21.*t31.*t34.*t198.*t199.*(1.0./2.0);
    t550 = L.*kappa_2.*t5.*t17.*t22.*t30.*t198.*t199.*w.*(1.0./2.0);
    t551 = L.*kappa_2.*t5.*t21.*t30.*t34.*t198.*t199.*w.*(1.0./2.0);
    t552 = L.*kappa_2.*t5.*t15.*t17.*t20.*t31.*t191.*w.*2.0;
    t553 = L.*kappa_2.*t5.*t15.*t19.*t23.*t30.*t191.*w.*2.0;
    t554 = kappa_2.*t3.*t5.*t10.*t22.*t25.*t31.*t198.*t199.*(1.0./2.0);
    t555 = L.*kappa_2.*t5.*t17.*t22.*t31.*t198.*t199.*w.*(1.0./2.0);
    t556 = L.*kappa_2.*t5.*t21.*t31.*t34.*t198.*t199.*w.*(1.0./2.0);
    t557 = L.*kappa_1.*kappa_2.*t5.*t17.*t24.*t34.*t191.*w.*3.0;
    t558 = L.*kappa_2.*t5.*t15.*t20.*t25.*t31.*t191.*w.*2.0;
    t559 = L.*kappa_2.*t5.*t15.*t23.*t30.*t34.*t191.*w.*2.0;
    t560 = L.*kappa_2.*t5.*t22.*t25.*t31.*t198.*t199.*w.*(1.0./2.0);
    t561 = L.*kappa_2.*t5.*t15.*t23.*t31.*t34.*t191.*w.*2.0;
    t562 = L.*kappa_2.*t3.*t5.*t15.*t19.*t21.*t30.*w.*2.0;
    t563 = L.*kappa_2.*t3.*t5.*t15.*t21.*t30.*t34.*w.*2.0;
    t564 = L.*kappa_2.*t3.*t5.*t15.*t21.*t31.*t34.*w.*2.0;
    t565 = kappa_1.*kappa_2.*t3.*t5.*t10.*t15.*t21.*t24.*t30.*t34;
    t566 = L.*kappa_1.*kappa_2.*t5.*t15.*t19.*t21.*t24.*t30.*w;
    t567 = kappa_1.*kappa_2.*t3.*t5.*t10.*t15.*t21.*t24.*t31.*t34;
    t568 = L.*kappa_1.*kappa_2.*t5.*t15.*t21.*t24.*t30.*t34.*w;
    t569 = L.*kappa_1.*kappa_2.*t5.*t15.*t21.*t24.*t31.*t34.*w;
    t570 = kappa_2.*t3.*t5.*t10.*t15.*t17.*t22.*t30.*t203.*t205;
    t571 = kappa_2.*t3.*t5.*t10.*t15.*t21.*t30.*t34.*t203.*t205;
    t572 = L.*kappa_2.*t3.*t5.*t17.*t20.*t30.*t198.*t199.*w;
    t573 = kappa_2.*t3.*t5.*t10.*t15.*t22.*t25.*t30.*t203.*t205;
    t574 = L.*kappa_2.*t5.*t15.*t17.*t22.*t30.*t203.*t205.*w;
    t575 = L.*kappa_2.*t5.*t15.*t21.*t30.*t34.*t203.*t205.*w;
    t576 = L.*kappa_2.*t3.*t5.*t17.*t20.*t31.*t198.*t199.*w;
    t577 = L.*kappa_2.*t3.*t5.*t19.*t23.*t30.*t198.*t199.*w;
    t578 = kappa_2.*t3.*t5.*t10.*t15.*t22.*t25.*t31.*t203.*t205;
    t579 = L.*kappa_2.*t5.*t15.*t22.*t25.*t30.*t203.*t205.*w;
    t580 = L.*kappa_2.*t3.*t5.*t20.*t25.*t31.*t198.*t199.*w;
    t581 = L.*kappa_2.*t3.*t5.*t23.*t30.*t34.*t198.*t199.*w;
    t582 = L.*kappa_2.*t5.*t15.*t22.*t25.*t31.*t203.*t205.*w;
    t583 = L.*kappa_2.*t3.*t5.*t23.*t31.*t34.*t198.*t199.*w;
    t584 = kappa_1.*kappa_2.*t2.*t5.*t17.*t20.*t24.*t30.*t198.*t199;
    t585 = kappa_1.*kappa_2.*t2.*t5.*t19.*t21.*t24.*t31.*t198.*t199;
    t586 = kappa_1.*kappa_2.*t2.*t5.*t20.*t24.*t25.*t30.*t198.*t199;
    t587 = kappa_1.*kappa_2.*t2.*t5.*t20.*t24.*t25.*t31.*t198.*t199;
    t588 = kappa_1.*kappa_2.*t5.*t10.*t15.*t17.*t22.*t24.*t30.*t191;
    t589 = kappa_1.*kappa_2.*t5.*t10.*t15.*t19.*t23.*t24.*t30.*t191;
    t590 = kappa_1.*kappa_2.*t5.*t10.*t15.*t22.*t24.*t25.*t30.*t191;
    t591 = kappa_1.*kappa_2.*t5.*t10.*t15.*t23.*t24.*t30.*t34.*t191;
    t592 = kappa_1.*kappa_2.*t5.*t10.*t15.*t22.*t24.*t25.*t31.*t191;
    t593 = kappa_1.*kappa_2.*t5.*t10.*t15.*t23.*t24.*t31.*t34.*t191;
    t594 = kappa_1.*kappa_2.*t3.*t5.*t10.*t15.*t19.*t21.*t24.*t30;
    t595 = L.*kappa_1.*kappa_2.*t3.*t5.*t15.*t23.*t24.*t30.*t34.*w.*2.0;
    t596 = L.*kappa_2.*t3.*t5.*t15.*t17.*t20.*t30.*t203.*t205.*w.*2.0;
    t597 = L.*kappa_1.*kappa_2.*t3.*t5.*t15.*t23.*t24.*t31.*t34.*w.*2.0;
    t598 = L.*kappa_2.*t3.*t5.*t15.*t20.*t25.*t30.*t203.*t205.*w.*2.0;
    t599 = L.*kappa_2.*t3.*t5.*t15.*t20.*t25.*t31.*t203.*t205.*w.*2.0;
    t600 = L.*kappa_2.*t3.*t5.*t15.*t23.*t30.*t34.*t203.*t205.*w.*2.0;
    t601 = kappa_1.*kappa_2.*t2.*t5.*t15.*t19.*t21.*t24.*t30.*t203.*t205.*2.0;
    t602 = kappa_1.*kappa_2.*t2.*t5.*t15.*t19.*t21.*t24.*t31.*t203.*t205.*2.0;
    t603 = kappa_1.*kappa_2.*t2.*t5.*t15.*t20.*t24.*t25.*t30.*t203.*t205.*2.0;
    t604 = kappa_1.*kappa_2.*t2.*t5.*t15.*t21.*t24.*t31.*t34.*t203.*t205.*2.0;
    t605 = kappa_1.*kappa_2.*t3.*t5.*t10.*t17.*t22.*t24.*t30.*t198.*t199.*(1.0./2.0);
    t606 = kappa_1.*kappa_2.*t3.*t5.*t10.*t19.*t23.*t24.*t30.*t198.*t199.*(1.0./2.0);
    t607 = L.*kappa_1.*kappa_2.*t5.*t15.*t17.*t20.*t24.*t30.*t191.*w.*2.0;
    t608 = kappa_1.*kappa_2.*t3.*t5.*t10.*t22.*t24.*t25.*t30.*t198.*t199.*(1.0./2.0);
    t609 = kappa_1.*kappa_2.*t3.*t5.*t10.*t23.*t24.*t30.*t34.*t198.*t199.*(1.0./2.0);
    t610 = L.*kappa_1.*kappa_2.*t5.*t17.*t22.*t24.*t30.*t198.*t199.*w.*(1.0./2.0);
    t611 = L.*kappa_1.*kappa_2.*t5.*t19.*t23.*t24.*t30.*t198.*t199.*w.*(1.0./2.0);
    t612 = L.*kappa_1.*kappa_2.*t5.*t15.*t19.*t21.*t24.*t31.*t191.*w.*2.0;
    t613 = L.*kappa_1.*kappa_2.*t5.*t15.*t20.*t24.*t25.*t30.*t191.*w.*2.0;
    t614 = kappa_1.*kappa_2.*t3.*t5.*t10.*t22.*t24.*t25.*t31.*t198.*t199.*(1.0./2.0);
    t615 = kappa_1.*kappa_2.*t3.*t5.*t10.*t23.*t24.*t31.*t34.*t198.*t199.*(1.0./2.0);
    t616 = L.*kappa_1.*kappa_2.*t5.*t22.*t24.*t25.*t30.*t198.*t199.*w.*(1.0./2.0);
    t617 = L.*kappa_1.*kappa_2.*t5.*t23.*t24.*t30.*t34.*t198.*t199.*w.*(1.0./2.0);
    t618 = L.*kappa_1.*kappa_2.*t5.*t15.*t20.*t24.*t25.*t31.*t191.*w.*2.0;
    t619 = L.*kappa_1.*kappa_2.*t5.*t22.*t24.*t25.*t31.*t198.*t199.*w.*(1.0./2.0);
    t620 = L.*kappa_1.*kappa_2.*t5.*t23.*t24.*t31.*t34.*t198.*t199.*w.*(1.0./2.0);
    t621 = L.*kappa_1.*kappa_2.*t3.*t5.*t15.*t19.*t23.*t24.*t30.*w.*2.0;
    t622 = L.*kappa_1.*kappa_2.*t3.*t5.*t17.*t20.*t24.*t30.*t198.*t199.*w;
    t623 = kappa_1.*kappa_2.*t3.*t5.*t10.*t15.*t22.*t24.*t25.*t30.*t203.*t205;
    t624 = kappa_1.*kappa_2.*t3.*t5.*t10.*t15.*t23.*t24.*t30.*t34.*t203.*t205;
    t625 = L.*kappa_1.*kappa_2.*t3.*t5.*t19.*t21.*t24.*t31.*t198.*t199.*w;
    t626 = L.*kappa_1.*kappa_2.*t3.*t5.*t20.*t24.*t25.*t30.*t198.*t199.*w;
    t627 = L.*kappa_1.*kappa_2.*t5.*t15.*t22.*t24.*t25.*t30.*t203.*t205.*w;
    t628 = L.*kappa_1.*kappa_2.*t5.*t15.*t23.*t24.*t30.*t34.*t203.*t205.*w;
    t629 = L.*kappa_1.*kappa_2.*t3.*t5.*t20.*t24.*t25.*t31.*t198.*t199.*w;
    t630 = L.*kappa_1.*kappa_2.*t3.*t5.*t15.*t19.*t21.*t24.*t30.*t203.*t205.*w.*2.0;
    t631 = L.*kappa_1.*kappa_2.*t3.*t5.*t15.*t19.*t21.*t24.*t31.*t203.*t205.*w.*2.0;
    t632 = L.*kappa_1.*kappa_2.*t3.*t5.*t15.*t20.*t24.*t25.*t30.*t203.*t205.*w.*2.0;
    t633 = L.*kappa_1.*kappa_2.*t3.*t5.*t15.*t21.*t24.*t31.*t34.*t203.*t205.*w.*2.0;
    t758 = t2.*t17.*t30.*2.0;
    t759 = t2.*t25.*t31.*2.0;
    t760 = t2.*t17.*t30.*t191.*2.0;
    t761 = t2.*t25.*t31.*t191.*2.0;
    t762 = t2.*t3.*t17.*t31.*2.0;
    t763 = t3.*t10.*t25.*t30;
    t764 = L.*t25.*t30.*w;
    t765 = L.*t25.*t30.*t191.*w.*3.0;
    t766 = t3.*t10.*t15.*t23.*t32;
    t767 = t3.*t10.*t15.*t23.*t33;
    t768 = L.*t15.*t23.*t32.*w;
    t769 = L.*t3.*t17.*t30.*w.*3.0;
    t770 = L.*t15.*t23.*t33.*w;
    t771 = L.*t3.*t25.*t31.*w.*3.0;
    t772 = kappa_1.*t2.*t24.*t25.*t30.*2.0;
    t773 = L.*t17.*t31.*t203.*t205.*w;
    t774 = kappa_2.*t2.*t5.*t17.*t19.*t191.*2.0;
    t775 = kappa_2.*t2.*t5.*t25.*t34.*t191.*2.0;
    t776 = kappa_1.*t2.*t24.*t25.*t30.*t191.*2.0;
    t777 = kappa_1.*t10.*t17.*t24.*t31.*t191;
    t778 = kappa_1.*t2.*t3.*t17.*t24.*t30.*2.0;
    t779 = kappa_1.*t2.*t3.*t24.*t25.*t31.*2.0;
    t780 = t2.*t3.*t25.*t30.*t203.*t205.*2.0;
    t781 = t3.*t10.*t17.*t31.*t203.*t205;
    t782 = kappa_1.*t2.*t21.*t24.*t32.*t198.*t199;
    t783 = kappa_1.*t2.*t21.*t24.*t33.*t198.*t199;
    t784 = L.*kappa_2.*t5.*t17.*t19.*t191.*w.*3.0;
    t785 = kappa_1.*t2.*t17.*t24.*t31.*t203.*t205.*2.0;
    t786 = L.*kappa_2.*t5.*t25.*t34.*t191.*w.*3.0;
    t787 = L.*kappa_1.*t3.*t24.*t25.*t30.*w.*3.0;
    t788 = kappa_2.*t2.*t5.*t15.*t19.*t21.*t31.*2.0;
    t789 = kappa_1.*t3.*t10.*t17.*t24.*t30.*t203.*t205;
    t790 = L.*kappa_1.*t15.*t21.*t24.*t32.*t191.*w.*2.0;
    t791 = L.*kappa_1.*t15.*t21.*t24.*t33.*t191.*w.*2.0;
    t792 = L.*kappa_1.*t17.*t24.*t30.*t203.*t205.*w;
    t793 = kappa_1.*t3.*t10.*t24.*t25.*t31.*t203.*t205;
    t794 = kappa_2.*t2.*t5.*t20.*t25.*t30.*t198.*t199;
    t795 = L.*kappa_1.*t24.*t25.*t31.*t203.*t205.*w;
    t796 = kappa_2.*t2.*t5.*t19.*t23.*t31.*t198.*t199;
    t797 = kappa_1.*kappa_2.*t2.*t5.*t19.*t24.*t25.*t191.*2.0;
    t798 = kappa_2.*t5.*t10.*t15.*t19.*t21.*t31.*t191;
    t799 = kappa_1.*kappa_2.*t5.*t10.*t17.*t24.*t34.*t191;
    t800 = kappa_2.*t5.*t10.*t15.*t22.*t25.*t30.*t191;
    t801 = kappa_2.*t3.*t5.*t10.*t15.*t19.*t23.*t30;
    t802 = kappa_2.*t3.*t5.*t10.*t15.*t23.*t30.*t34;
    t803 = L.*kappa_2.*t5.*t15.*t19.*t23.*t30.*w;
    t804 = kappa_2.*t3.*t5.*t10.*t15.*t23.*t31.*t34;
    t805 = L.*kappa_2.*t5.*t15.*t23.*t30.*t34.*w;
    t806 = L.*kappa_2.*t5.*t15.*t23.*t31.*t34.*w;
    t807 = L.*kappa_1.*t3.*t21.*t24.*t33.*t198.*t199.*w;
    t808 = kappa_1.*kappa_2.*t2.*t5.*t15.*t19.*t23.*t24.*t31.*2.0;
    t809 = L.*kappa_1.*t3.*t17.*t24.*t31.*t203.*t205.*w.*3.0;
    t810 = kappa_2.*t2.*t5.*t15.*t17.*t20.*t31.*t203.*t205.*2.0;
    t811 = kappa_2.*t2.*t5.*t15.*t19.*t23.*t30.*t203.*t205.*2.0;
    t812 = kappa_2.*t2.*t5.*t15.*t19.*t23.*t31.*t203.*t205.*2.0;
    t813 = kappa_2.*t2.*t5.*t15.*t23.*t31.*t34.*t203.*t205.*2.0;
    t814 = kappa_2.*t3.*t5.*t10.*t19.*t21.*t31.*t198.*t199.*(1.0./2.0);
    t815 = kappa_2.*t3.*t5.*t10.*t22.*t25.*t30.*t198.*t199.*(1.0./2.0);
    t816 = L.*kappa_2.*t5.*t19.*t21.*t31.*t198.*t199.*w.*(1.0./2.0);
    t817 = L.*kappa_2.*t5.*t15.*t20.*t25.*t30.*t191.*w.*2.0;
    t818 = L.*kappa_2.*t5.*t22.*t25.*t30.*t198.*t199.*w.*(1.0./2.0);
    t819 = L.*kappa_1.*kappa_2.*t5.*t19.*t24.*t25.*t191.*w.*3.0;
    t820 = L.*kappa_2.*t5.*t15.*t19.*t23.*t31.*t191.*w.*2.0;
    t821 = L.*kappa_2.*t3.*t5.*t15.*t19.*t21.*t31.*w.*2.0;
    t822 = L.*kappa_1.*t3.*t21.*t24.*t32.*t198.*t199.*w;
    t823 = kappa_1.*kappa_2.*t3.*t5.*t10.*t15.*t19.*t21.*t24.*t31;
    t824 = L.*kappa_1.*kappa_2.*t5.*t15.*t19.*t21.*t24.*t31.*w;
    t825 = kappa_2.*t3.*t5.*t10.*t15.*t19.*t21.*t30.*t203.*t205;
    t826 = kappa_2.*t3.*t5.*t10.*t15.*t19.*t21.*t31.*t203.*t205;
    t827 = L.*kappa_2.*t5.*t15.*t19.*t21.*t30.*t203.*t205.*w;
    t828 = kappa_2.*t3.*t5.*t10.*t15.*t17.*t22.*t31.*t203.*t205;
    t829 = kappa_2.*t3.*t5.*t10.*t15.*t21.*t31.*t34.*t203.*t205;
    t830 = L.*kappa_2.*t5.*t15.*t19.*t21.*t31.*t203.*t205.*w;
    t831 = L.*kappa_2.*t3.*t5.*t20.*t25.*t30.*t198.*t199.*w;
    t832 = L.*kappa_2.*t5.*t15.*t17.*t22.*t31.*t203.*t205.*w;
    t833 = L.*kappa_2.*t5.*t15.*t21.*t31.*t34.*t203.*t205.*w;
    t834 = L.*kappa_2.*t3.*t5.*t19.*t23.*t31.*t198.*t199.*w;
    t835 = kappa_1.*kappa_2.*t2.*t5.*t19.*t21.*t24.*t30.*t198.*t199;
    t836 = kappa_1.*kappa_2.*t2.*t5.*t17.*t20.*t24.*t31.*t198.*t199;
    t837 = kappa_1.*kappa_2.*t2.*t5.*t21.*t24.*t30.*t34.*t198.*t199;
    t838 = kappa_1.*kappa_2.*t2.*t5.*t21.*t24.*t31.*t34.*t198.*t199;
    t839 = kappa_1.*kappa_2.*t5.*t10.*t15.*t17.*t22.*t24.*t31.*t191;
    t840 = kappa_1.*kappa_2.*t5.*t10.*t15.*t19.*t23.*t24.*t31.*t191;
    t841 = L.*kappa_1.*kappa_2.*t3.*t5.*t15.*t19.*t23.*t24.*t31.*w.*2.0;
    t842 = L.*kappa_2.*t3.*t5.*t15.*t17.*t20.*t31.*t203.*t205.*w.*2.0;
    t843 = L.*kappa_2.*t3.*t5.*t15.*t19.*t23.*t30.*t203.*t205.*w.*2.0;
    t844 = L.*kappa_2.*t3.*t5.*t15.*t19.*t23.*t31.*t203.*t205.*w.*2.0;
    t845 = L.*kappa_2.*t3.*t5.*t15.*t23.*t31.*t34.*t203.*t205.*w.*2.0;
    t846 = kappa_1.*kappa_2.*t2.*t5.*t15.*t17.*t20.*t24.*t30.*t203.*t205.*2.0;
    t847 = kappa_1.*kappa_2.*t2.*t5.*t15.*t17.*t20.*t24.*t31.*t203.*t205.*2.0;
    t848 = kappa_1.*kappa_2.*t2.*t5.*t15.*t21.*t24.*t30.*t34.*t203.*t205.*2.0;
    t849 = kappa_1.*kappa_2.*t2.*t5.*t15.*t20.*t24.*t25.*t31.*t203.*t205.*2.0;
    t850 = L.*kappa_1.*kappa_2.*t5.*t15.*t19.*t21.*t24.*t30.*t191.*w.*2.0;
    t851 = kappa_1.*kappa_2.*t3.*t5.*t10.*t17.*t22.*t24.*t31.*t198.*t199.*(1.0./2.0);
    t852 = kappa_1.*kappa_2.*t3.*t5.*t10.*t19.*t23.*t24.*t31.*t198.*t199.*(1.0./2.0);
    t853 = L.*kappa_1.*kappa_2.*t5.*t15.*t17.*t20.*t24.*t31.*t191.*w.*2.0;
    t854 = L.*kappa_1.*kappa_2.*t5.*t15.*t21.*t24.*t30.*t34.*t191.*w.*2.0;
    t855 = L.*kappa_1.*kappa_2.*t5.*t17.*t22.*t24.*t31.*t198.*t199.*w.*(1.0./2.0);
    t856 = L.*kappa_1.*kappa_2.*t5.*t19.*t23.*t24.*t31.*t198.*t199.*w.*(1.0./2.0);
    t857 = L.*kappa_1.*kappa_2.*t5.*t15.*t21.*t24.*t31.*t34.*t191.*w.*2.0;
    t858 = kappa_1.*kappa_2.*t3.*t5.*t10.*t15.*t17.*t22.*t24.*t30.*t203.*t205;
    t859 = kappa_1.*kappa_2.*t3.*t5.*t10.*t15.*t19.*t23.*t24.*t30.*t203.*t205;
    t860 = L.*kappa_1.*kappa_2.*t3.*t5.*t19.*t21.*t24.*t30.*t198.*t199.*w;
    t861 = kappa_1.*kappa_2.*t3.*t5.*t10.*t15.*t17.*t22.*t24.*t31.*t203.*t205;
    t862 = kappa_1.*kappa_2.*t3.*t5.*t10.*t15.*t19.*t23.*t24.*t31.*t203.*t205;
    t863 = L.*kappa_1.*kappa_2.*t5.*t15.*t17.*t22.*t24.*t30.*t203.*t205.*w;
    t864 = L.*kappa_1.*kappa_2.*t5.*t15.*t19.*t23.*t24.*t30.*t203.*t205.*w;
    t865 = L.*kappa_1.*kappa_2.*t3.*t5.*t17.*t20.*t24.*t31.*t198.*t199.*w;
    t866 = L.*kappa_1.*kappa_2.*t3.*t5.*t21.*t24.*t30.*t34.*t198.*t199.*w;
    t867 = kappa_1.*kappa_2.*t3.*t5.*t10.*t15.*t22.*t24.*t25.*t31.*t203.*t205;
    t868 = kappa_1.*kappa_2.*t3.*t5.*t10.*t15.*t23.*t24.*t31.*t34.*t203.*t205;
    t869 = L.*kappa_1.*kappa_2.*t5.*t15.*t17.*t22.*t24.*t31.*t203.*t205.*w;
    t870 = L.*kappa_1.*kappa_2.*t5.*t15.*t19.*t23.*t24.*t31.*t203.*t205.*w;
    t871 = L.*kappa_1.*kappa_2.*t3.*t5.*t21.*t24.*t31.*t34.*t198.*t199.*w;
    t872 = L.*kappa_1.*kappa_2.*t5.*t15.*t22.*t24.*t25.*t31.*t203.*t205.*w;
    t873 = L.*kappa_1.*kappa_2.*t5.*t15.*t23.*t24.*t31.*t34.*t203.*t205.*w;
    t874 = L.*kappa_1.*kappa_2.*t3.*t5.*t15.*t17.*t20.*t24.*t30.*t203.*t205.*w.*2.0;
    t875 = L.*kappa_1.*kappa_2.*t3.*t5.*t15.*t17.*t20.*t24.*t31.*t203.*t205.*w.*2.0;
    t876 = L.*kappa_1.*kappa_2.*t3.*t5.*t15.*t21.*t24.*t30.*t34.*t203.*t205.*w.*2.0;
    t877 = L.*kappa_1.*kappa_2.*t3.*t5.*t15.*t20.*t24.*t25.*t31.*t203.*t205.*w.*2.0;
    t634 = -t83+t84-t88-t90+t93-t94-t96+t98-t99-t100+t102-t103+t104-t107+t108+t109-...
            t111+t112+t113-t115+t116+t117+t118-t119-t164-t170-t172+t173-t175+t178+t179+...
            t182-t207-t208-t209-t210-t211-t212-t213-t214-t215-t216-t217+t342+t343+t344+...
            t345+t346+t349+t353+t355+t357+t458+t459+t460+t461+t462+t463+t464+t465+t466+...
            t467+t468+t469+t470+t471+t472+t473+t474+t475+t476+t477+t478+t479+t480+t481+...
            t482+t483+t484+t485+t486+t487+t488+t489+t490+t491+t492+t493+t494+t495+t496+...
            t497+t498+t499+t500+t501+t502+t503+t504+t505+t506+t507+t508+t509+t510+t511+...
            t512+t513+t514+t515+t516+t517+t518+t519+t520+t521+t522+t523+t524+t525+t526+...
            t527+t528+t529+t530+t531+t532+t533+t534+t535+t536+t537+t538+t539+t540+t541+...
            t542+t543+t544+t545+t546+t547+t548+t549+t550+t551+t552+t553+t554+t555+t556+...
            t557+t558+t559+t560+t561+t562+t563+t564+t565+t566+t567+t568+t569+t570+t571+...
            t572+t573+t574+t575+t576+t577+t578+t579+t580+t581+t582+t583+t584+t585+t586+...
            t587+t588+t589+t590+t591+t592+t593+t594+t595+t596+t597+t598+t599+t600+t601+...
            t602+t603+t604+t605+t606+t607+t608+t609+t610+t611+t612+t613+t614+t615+t616+...
            t617+t618+t619+t620+t621+t622+t623+t624+t625+t626+t627+t628+t629+t630+t631+...
            t632+t633-t758-t759-t760-t761-t762-t763-t764-t765-t766-t767-t768-t769-t770-...
            t771-t772-t773-t774-t775-t776-t777-t778-t779-t780-t781-t782-t783-t784-t785-...
            t786-t787-t788-t789-t790-t791-t792-t793-t794-t795-t796-t797-t798-t799-t800-...
            t801-t802-t803-t804-t805-t806-t807-t808-t809-t810-t811-t812-t813-t814-t815-...
            t816-t817-t818-t819-t820-t821-t822-t823-t824-t825-t826-t827-t828-t829-t830-...
            t831-t832-t833-t834-t835-t836-t837-t838-t839-t840-t841-t842-t843-t844-t845-...
            t846-t847-t848-t849-t850-t851-t852-t853-t854-t855-t856-t857-t858-t859-t860-...
            t861-t862-t863-t864-t865-t866-t867-t868-t869-t870-t871-t872-t873-t874-t875-t876-t877;
    t884 = kappa_2.*t2.*t5.*t15.*t17.*t22.*t30.*2.0;
    t885 = kappa_2.*t2.*t5.*t15.*t17.*t22.*t31.*2.0;
    t886 = kappa_2.*t2.*t5.*t15.*t22.*t25.*t31.*2.0;
    t887 = kappa_2.*t3.*t5.*t10.*t15.*t20.*t25.*t30;
    t888 = L.*kappa_2.*t5.*t15.*t20.*t25.*t30.*w;
    t889 = kappa_1.*kappa_2.*t2.*t5.*t15.*t17.*t22.*t24.*t30.*2.0;
    t890 = kappa_1.*kappa_2.*t2.*t5.*t15.*t22.*t24.*t25.*t30.*2.0;
    t891 = kappa_1.*kappa_2.*t2.*t5.*t15.*t22.*t24.*t25.*t31.*2.0;
    t892 = L.*kappa_2.*t3.*t5.*t15.*t17.*t22.*t30.*w.*2.0;
    t893 = L.*kappa_2.*t3.*t5.*t15.*t17.*t22.*t31.*w.*2.0;
    t894 = L.*kappa_2.*t3.*t5.*t15.*t22.*t25.*t31.*w.*2.0;
    t895 = kappa_1.*kappa_2.*t3.*t5.*t10.*t15.*t17.*t20.*t24.*t31;
    t896 = L.*kappa_1.*kappa_2.*t5.*t15.*t17.*t20.*t24.*t31.*w;
    t897 = L.*kappa_1.*kappa_2.*t3.*t5.*t15.*t22.*t24.*t25.*t30.*w.*2.0;
    t898 = L.*kappa_1.*kappa_2.*t3.*t5.*t15.*t22.*t24.*t25.*t31.*w.*2.0;
    t899 = L.*kappa_1.*kappa_2.*t3.*t5.*t15.*t17.*t22.*t24.*t30.*w.*2.0;
    t635 = t35-t36+t37+t38-t39+t40+t41-t42+t43-t44+t45-t46+t47+t48-t49+t50+t51-...
           t52+t53-t54+t87+t91+t95+t101+t106+t110+t114+t120-t174-t177-t180-t181+...
           t207+t208+t209+t210+t211+t212+t213+t214+t215+t216+t217-t342-t343-t344-...
           t345-t346+t347+t348-t349+t350+t351+t352-t353+t354-t355+t356-t357+t358+...
           t359+t360+t361+t362+t363+t364+t365+t366-t884-t885-t886-t887-t888-t889-...
           t890-t891-t892-t893-t894-t895-t896-t897-t898-t899;
    t636 = t17.*t31;
    t637 = kappa_1.*t17.*t24.*t30;
    t638 = kappa_1.*t24.*t25.*t31;
    t639 = kappa_1.*kappa_2.*t5.*t17.*t24.*t34;
    t672 = t25.*t30;
    t673 = kappa_2.*t5.*t17.*t19;
    t674 = kappa_2.*t5.*t25.*t34;
    t675 = kappa_1.*kappa_2.*t5.*t19.*t24.*t25;
    t640 = t636+t637+t638+t639-t672-t673-t674-t675;
    t755 = kappa_2.*t5.*t17.*t34;
    t756 = kappa_1.*kappa_2.*t5.*t17.*t19.*t24;
    t757 = kappa_1.*kappa_2.*t5.*t24.*t25.*t34;
    t878 = 1.0./L.^2;
    t879 = 1.0./t191;
    t880 = t17.^2;
    t881 = t25.^2;
    t882 = kappa_1.*t24;
    t883 = t882+1.0;
    t900 = t3.*t10.*t880;
    t901 = t3.*t10.*t881;
    t902 = L.*t880.*w;
    t903 = L.*t881.*w;
    t904 = t2.*t15.*t17.*t21.*t31.*2.0;
    t905 = t2.*t15.*t17.*t23.*t30.*2.0;
    t906 = t2.*t15.*t23.*t25.*t31.*2.0;
    t907 = kappa_2.*t2.*t5.*t15.*t20.*t880.*2.0;
    t908 = kappa_2.*t2.*t5.*t15.*t20.*t881.*2.0;
    t909 = t3.*t10.*t15.*t17.*t21.*t30;
    t910 = L.*t15.*t17.*t21.*t30.*w;
    t911 = t3.*t10.*t15.*t21.*t25.*t31;
    t912 = t3.*t10.*t15.*t23.*t25.*t30;
    t913 = L.*t15.*t21.*t25.*t31.*w;
    t914 = L.*t15.*t23.*t25.*t30.*w;
    t915 = kappa_2.*t3.*t5.*t10.*t15.*t22.*t880;
    t916 = kappa_2.*t3.*t5.*t10.*t15.*t22.*t881;
    t917 = L.*kappa_2.*t5.*t15.*t22.*t880.*w;
    t918 = L.*t3.*t15.*t17.*t21.*t31.*w.*2.0;
    t919 = L.*t3.*t15.*t17.*t23.*t30.*w.*2.0;
    t920 = L.*kappa_2.*t5.*t15.*t22.*t881.*w;
    t921 = L.*t3.*t15.*t23.*t25.*t31.*w.*2.0;
    t922 = kappa_2.*t2.*t5.*t15.*t17.*t23.*t34.*2.0;
    t923 = L.*kappa_2.*t3.*t5.*t15.*t20.*t880.*w.*2.0;
    t924 = L.*kappa_2.*t3.*t5.*t15.*t20.*t881.*w.*2.0;
    t925 = kappa_2.*t3.*t5.*t10.*t15.*t17.*t19.*t23;
    t926 = kappa_2.*t3.*t5.*t10.*t15.*t17.*t21.*t34;
    t927 = L.*kappa_2.*t5.*t15.*t17.*t19.*t23.*w;
    t928 = L.*kappa_2.*t5.*t15.*t17.*t21.*t34.*w;
    t929 = kappa_2.*t3.*t5.*t10.*t15.*t23.*t25.*t34;
    t930 = L.*kappa_2.*t5.*t15.*t23.*t25.*t34.*w;
    t931 = L.*kappa_2.*t3.*t5.*t15.*t17.*t23.*t34.*w.*2.0;
    t933 = t2.*t3.*t880.*2.0;
    t934 = t2.*t3.*t881.*2.0;
    t935 = t2.*t15.*t21.*t25.*t30.*2.0;
    t936 = t3.*t10.*t15.*t17.*t23.*t31;
    t937 = L.*t15.*t17.*t23.*t31.*w;
    t938 = L.*t3.*t15.*t21.*t25.*t30.*w.*2.0;
    t939 = kappa_2.*t2.*t5.*t15.*t17.*t19.*t21.*2.0;
    t940 = kappa_2.*t2.*t5.*t15.*t19.*t23.*t25.*2.0;
    t941 = kappa_2.*t2.*t5.*t15.*t21.*t25.*t34.*2.0;
    t942 = kappa_2.*t3.*t5.*t10.*t15.*t19.*t21.*t25;
    t943 = L.*kappa_2.*t5.*t15.*t19.*t21.*t25.*w;
    t944 = L.*kappa_2.*t3.*t5.*t15.*t17.*t19.*t21.*w.*2.0;
    t945 = L.*kappa_2.*t3.*t5.*t15.*t19.*t23.*t25.*w.*2.0;
    t946 = L.*kappa_2.*t3.*t5.*t15.*t21.*t25.*t34.*w.*2.0;
    t932 = t900+t901+t902+t903+t904+t905+t906+t907+t908+t909+t910+t911+t912+t913+t914+ ...
           t915+t916+t917+t918+t919+t920+t921+t922+t923+t924+t925+t926+t927+t928+t929+ ...
           t930+t931-t933-t934-t935-t936-t937-t938-t939-t940-t941-t942-t943-t944-t945-t946;
    
    dC_1delta = reshape([0.0,0.0,0.0,...
                         deltap_i.*(t195.*t878.*t879-t3.*t13.*t878.*t879.*2.0), ...
                         0.0,0.0,0.0,0.0,0.0,dalpha_2.*(t184.*(R.*kappa_2.*t2.*t15.*t17.*t20.*t122.*2.0+R.*kappa_2.*t2.*t15.*t23.*t34.*t122.*2.0+L.*R.*kappa_2.*t15.*t17.*t22.*t122.*w+L.*R.*kappa_2.*t15.*t21.*t34.*t122.*w+R.*kappa_2.*t3.*t10.*t15.*t17.*t22.*t122+R.*kappa_2.*t3.*t10.*t15.*t21.*t34.*t122+L.*R.*kappa_2.*t3.*t15.*t17.*t20.*t122.*w.*2.0+L.*R.*kappa_2.*t3.*t15.*t23.*t34.*t122.*w.*2.0+R.*kappa_1.*kappa_2.*t2.*t15.*t20.*t24.*t25.*t122.*2.0-R.*kappa_1.*kappa_2.*t2.*t15.*t21.*t24.*t34.*t122.*2.0+L.*R.*kappa_1.*kappa_2.*t15.*t22.*t24.*t25.*t122.*w+L.*R.*kappa_1.*kappa_2.*t15.*t23.*t24.*t34.*t122.*w+R.*kappa_1.*kappa_2.*t3.*t10.*t15.*t22.*t24.*t25.*t122+R.*kappa_1.*kappa_2.*t3.*t10.*t15.*t23.*t24.*t34.*t122+L.*R.*kappa_1.*kappa_2.*t3.*t15.*t20.*t24.*t25.*t122.*w.*2.0-L.*R.*kappa_1.*kappa_2.*t3.*t15.*t21.*t24.*t34.*t122.*w.*2.0)-t148.*t183.*t420)+deltap_i.*(t184.*(t220+t221+t222+t227+t228+t230+t232-R.*t3.*t10.*t25-R.*t2.*t17.*t191.*2.0+R.*t10.*t17.*t191-L.*R.*t25.*w+R.*t2.*t15.*t21.*t30.*2.0-L.*R.*t15.*t23.*t30.*w-R.*kappa_1.*t2.*t3.*t17.*t24.*2.0-R.*kappa_1.*t2.*t24.*t25.*t191.*2.0+R.*kappa_1.*t10.*t24.*t25.*t191-R.*t3.*t10.*t15.*t23.*t30+R.*t10.*t15.*t21.*t30.*t191+R.*t2.*t23.*t30.*t198.*t199+L.*R.*t3.*t15.*t21.*t30.*w.*2.0+L.*R.*t15.*t23.*t30.*t191.*w.*2.0+L.*R.*t21.*t30.*t198.*t199.*w.*(1.0./2.0)-R.*kappa_2.*t2.*t5.*t15.*t20.*t25.*2.0+R.*kappa_2.*t2.*t5.*t15.*t21.*t34.*2.0+R.*kappa_1.*t2.*t15.*t23.*t24.*t30.*2.0+R.*t3.*t10.*t21.*t30.*t198.*t199.*(1.0./2.0)-R.*t2.*t15.*t23.*t31.*t203.*t205.*2.0-L.*R.*kappa_2.*t5.*t15.*t22.*t25.*w-L.*R.*kappa_2.*t5.*t15.*t23.*t34.*w+L.*R.*kappa_1.*t15.*t21.*t24.*t30.*w+L.*R.*t3.*t23.*t30.*t198.*t199.*w-L.*R.*t15.*t21.*t31.*t203.*t205.*w-R.*kappa_2.*t3.*t5.*t10.*t15.*t22.*t25-R.*kappa_2.*t3.*t5.*t10.*t15.*t23.*t34+R.*kappa_1.*t3.*t10.*t15.*t21.*t24.*t30+R.*kappa_2.*t5.*t10.*t15.*t17.*t22.*t191+R.*kappa_2.*t5.*t10.*t15.*t21.*t34.*t191+R.*kappa_1.*t10.*t15.*t23.*t24.*t30.*t191+R.*kappa_2.*t2.*t5.*t17.*t20.*t198.*t199+R.*kappa_2.*t2.*t5.*t23.*t34.*t198.*t199-R.*kappa_1.*t2.*t21.*t24.*t30.*t198.*t199-R.*t3.*t10.*t15.*t21.*t31.*t203.*t205-L.*R.*kappa_2.*t3.*t5.*t15.*t20.*t25.*w.*2.0+L.*R.*kappa_2.*t3.*t5.*t15.*t21.*t34.*w.*2.0+L.*R.*kappa_1.*t3.*t15.*t23.*t24.*t30.*w.*2.0+L.*R.*kappa_2.*t5.*t15.*t17.*t20.*t191.*w.*2.0+L.*R.*kappa_2.*t5.*t15.*t23.*t34.*t191.*w.*2.0-L.*R.*kappa_1.*t15.*t21.*t24.*t30.*t191.*w.*2.0+L.*R.*kappa_2.*t5.*t17.*t22.*t198.*t199.*w.*(1.0./2.0)+L.*R.*kappa_2.*t5.*t21.*t34.*t198.*t199.*w.*(1.0./2.0)+L.*R.*kappa_1.*t23.*t24.*t30.*t198.*t199.*w.*(1.0./2.0)-L.*R.*t3.*t15.*t23.*t31.*t203.*t205.*w.*2.0+R.*kappa_1.*kappa_2.*t2.*t5.*t15.*t23.*t24.*t34.*2.0+R.*kappa_2.*t3.*t5.*t10.*t17.*t22.*t198.*t199.*(1.0./2.0)+R.*kappa_2.*t3.*t5.*t10.*t21.*t34.*t198.*t199.*(1.0./2.0)+R.*kappa_1.*t3.*t10.*t23.*t24.*t30.*t198.*t199.*(1.0./2.0)+R.*kappa_1.*t2.*t15.*t21.*t24.*t31.*t203.*t205.*2.0+L.*R.*kappa_1.*kappa_2.*t5.*t15.*t21.*t24.*t34.*w+L.*R.*kappa_2.*t3.*t5.*t17.*t20.*t198.*t199.*w+L.*R.*kappa_2.*t3.*t5.*t23.*t34.*t198.*t199.*w-L.*R.*kappa_1.*t3.*t21.*t24.*t30.*t198.*t199.*w-L.*R.*kappa_1.*t15.*t23.*t24.*t31.*t203.*t205.*w+R.*kappa_1.*kappa_2.*t3.*t5.*t10.*t15.*t21.*t24.*t34+R.*kappa_1.*kappa_2.*t5.*t10.*t15.*t22.*t24.*t25.*t191+R.*kappa_1.*kappa_2.*t5.*t10.*t15.*t23.*t24.*t34.*t191+R.*kappa_1.*kappa_2.*t2.*t5.*t20.*t24.*t25.*t198.*t199-R.*kappa_1.*kappa_2.*t2.*t5.*t21.*t24.*t34.*t198.*t199-R.*kappa_1.*t3.*t10.*t15.*t23.*t24.*t31.*t203.*t205+L.*R.*kappa_1.*kappa_2.*t3.*t5.*t15.*t23.*t24.*t34.*w.*2.0+L.*R.*kappa_1.*kappa_2.*t5.*t15.*t20.*t24.*t25.*t191.*w.*2.0-L.*R.*kappa_1.*kappa_2.*t5.*t15.*t21.*t24.*t34.*t191.*w.*2.0+L.*R.*kappa_1.*kappa_2.*t5.*t22.*t24.*t25.*t198.*t199.*w.*(1.0./2.0)+L.*R.*kappa_1.*kappa_2.*t5.*t23.*t24.*t34.*t198.*t199.*w.*(1.0./2.0)+L.*R.*kappa_1.*t3.*t15.*t21.*t24.*t31.*t203.*t205.*w.*2.0+R.*kappa_1.*kappa_2.*t3.*t5.*t10.*t22.*t24.*t25.*t198.*t199.*(1.0./2.0)+R.*kappa_1.*kappa_2.*t3.*t5.*t10.*t23.*t24.*t34.*t198.*t199.*(1.0./2.0)+L.*R.*kappa_1.*kappa_2.*t3.*t5.*t20.*t24.*t25.*t198.*t199.*w-L.*R.*kappa_1.*kappa_2.*t3.*t5.*t21.*t24.*t34.*t198.*t199.*w)-t148.*t183.*t634)+dkappa_2.*(t184.*(R.*t2.*t5.*t15.*t17.*t20.*2.0+R.*t2.*t5.*t15.*t23.*t34.*2.0+L.*R.*t5.*t15.*t17.*t22.*w+L.*R.*t5.*t15.*t21.*t34.*w+R.*t3.*t5.*t10.*t15.*t17.*t22+R.*t3.*t5.*t10.*t15.*t21.*t34+L.*R.*t3.*t5.*t15.*t17.*t20.*w.*2.0+L.*R.*t3.*t5.*t15.*t23.*t34.*w.*2.0+R.*kappa_1.*t2.*t5.*t15.*t20.*t24.*t25.*2.0-R.*kappa_1.*t2.*t5.*t15.*t21.*t24.*t34.*2.0+L.*R.*kappa_1.*t5.*t15.*t22.*t24.*t25.*w+L.*R.*kappa_1.*t5.*t15.*t23.*t24.*t34.*w+R.*kappa_1.*t3.*t5.*t10.*t15.*t22.*t24.*t25+R.*kappa_1.*t3.*t5.*t10.*t15.*t23.*t24.*t34+L.*R.*kappa_1.*t3.*t5.*t15.*t20.*t24.*t25.*w.*2.0-L.*R.*kappa_1.*t3.*t5.*t15.*t21.*t24.*t34.*w.*2.0)-t148.*t183.*t288)+dkappa_1.*(t184.*(L.*R.*t24.*t25.*w-R.*t2.*t3.*t24.*t25.*2.0+R.*t3.*t10.*t24.*t25-R.*t2.*t15.*t21.*t24.*t30.*2.0+L.*R.*t15.*t23.*t24.*t30.*w+R.*t3.*t10.*t15.*t23.*t24.*t30-L.*R.*t3.*t15.*t21.*t24.*t30.*w.*2.0+R.*kappa_2.*t2.*t5.*t15.*t20.*t24.*t25.*2.0-R.*kappa_2.*t2.*t5.*t15.*t21.*t24.*t34.*2.0+L.*R.*kappa_2.*t5.*t15.*t22.*t24.*t25.*w+L.*R.*kappa_2.*t5.*t15.*t23.*t24.*t34.*w+R.*kappa_2.*t3.*t5.*t10.*t15.*t22.*t24.*t25+R.*kappa_2.*t3.*t5.*t10.*t15.*t23.*t24.*t34+L.*R.*kappa_2.*t3.*t5.*t15.*t20.*t24.*t25.*w.*2.0-L.*R.*kappa_2.*t3.*t5.*t15.*t21.*t24.*t34.*w.*2.0)-t148.*t183.*t457)+dalpha_1.*(t184.*(L.*R.*kappa_1.*t25.*t219.*w-R.*kappa_1.*t2.*t3.*t25.*t219.*2.0+R.*kappa_1.*t3.*t10.*t25.*t219-R.*kappa_1.*t2.*t15.*t21.*t30.*t219.*2.0+L.*R.*kappa_1.*t15.*t23.*t30.*t219.*w+R.*kappa_1.*t3.*t10.*t15.*t23.*t30.*t219-L.*R.*kappa_1.*t3.*t15.*t21.*t30.*t219.*w.*2.0+R.*kappa_1.*kappa_2.*t2.*t5.*t15.*t20.*t25.*t219.*2.0-R.*kappa_1.*kappa_2.*t2.*t5.*t15.*t21.*t34.*t219.*2.0+L.*R.*kappa_1.*kappa_2.*t5.*t15.*t22.*t25.*t219.*w+L.*R.*kappa_1.*kappa_2.*t5.*t15.*t23.*t34.*t219.*w+R.*kappa_1.*kappa_2.*t3.*t5.*t10.*t15.*t22.*t25.*t219+R.*kappa_1.*kappa_2.*t3.*t5.*t10.*t15.*t23.*t34.*t219+L.*R.*kappa_1.*kappa_2.*t3.*t5.*t15.*t20.*t25.*t219.*w.*2.0-L.*R.*kappa_1.*kappa_2.*t3.*t5.*t15.*t21.*t34.*t219.*w.*2.0)-t148.*t183.*t341)+deltap_o.*((t223+t224+t225+t226+t229+t231-R.*kappa_2.*t2.*t5.*t15.*t17.*t22.*2.0+L.*R.*kappa_2.*t5.*t15.*t17.*t20.*w+R.*kappa_2.*t3.*t5.*t10.*t15.*t17.*t20-L.*R.*kappa_2.*t3.*t5.*t15.*t17.*t22.*w.*2.0-R.*kappa_1.*kappa_2.*t2.*t5.*t15.*t19.*t21.*t24.*2.0-R.*kappa_1.*kappa_2.*t2.*t5.*t15.*t22.*t24.*t25.*2.0+L.*R.*kappa_1.*kappa_2.*t5.*t15.*t20.*t24.*t25.*w+R.*kappa_1.*kappa_2.*t3.*t5.*t10.*t15.*t20.*t24.*t25-L.*R.*kappa_1.*kappa_2.*t3.*t5.*t15.*t19.*t21.*t24.*w.*2.0-L.*R.*kappa_1.*kappa_2.*t3.*t5.*t15.*t22.*t24.*t25.*w.*2.0)./(t35+t36+t37+t38+t39+t40+t41+t42+t43+t44+t45+t46+t47+t48+t49+t50+t51+t52+t53+t54+t55+t56+t57+t58+t59+t60+t61+t62+t63+t64+t65+t66+t67+t68+t69+t70+t71+t72+t73+t74+t75+t76+t77+t78+t79+t80+t81+t82+t83+t84+t85+t86+t88+t89+t90+t92+t93+t94+t96+t97+t98+t99+t100+t102+t103+t104+t105+t107+t108+t109+t111+t112+t113+t115+t116+t117+t118+t119-t2.*t25.*t30.*2.0-t2.*t3.*t17.*t30.*2.0-t2.*t3.*t25.*t31.*2.0-L.*t3.*t25.*t30.*w.*3.0-kappa_2.*t2.*t5.*t17.*t19.*2.0-kappa_2.*t2.*t5.*t25.*t34.*2.0-kappa_2.*t2.*t3.*t5.*t17.*t19.*2.0-kappa_2.*t2.*t3.*t5.*t25.*t34.*2.0-kappa_1.*t2.*t3.*t24.*t25.*t30.*2.0-kappa_1.*t3.*t10.*t17.*t24.*t31-kappa_1.*t2.*t15.*t21.*t24.*t32.*2.0-kappa_1.*t2.*t15.*t21.*t24.*t33.*2.0-L.*kappa_1.*t17.*t24.*t31.*w-L.*kappa_2.*t3.*t5.*t17.*t19.*w.*3.0-L.*kappa_2.*t3.*t5.*t25.*t34.*w.*3.0-kappa_1.*kappa_2.*t2.*t5.*t19.*t24.*t25.*2.0-kappa_2.*t2.*t5.*t15.*t19.*t23.*t31.*2.0-kappa_2.*t2.*t5.*t15.*t20.*t25.*t30.*2.0-L.*kappa_1.*kappa_2.*t5.*t17.*t24.*t34.*w-L.*kappa_2.*t5.*t15.*t19.*t21.*t31.*w-L.*kappa_1.*t3.*t15.*t21.*t24.*t32.*w.*2.0-L.*kappa_1.*t3.*t15.*t21.*t24.*t33.*w.*2.0-L.*kappa_2.*t5.*t15.*t22.*t25.*t30.*w-kappa_1.*kappa_2.*t2.*t3.*t5.*t19.*t24.*t25.*2.0-kappa_1.*kappa_2.*t3.*t5.*t10.*t17.*t24.*t34-kappa_2.*t3.*t5.*t10.*t15.*t19.*t21.*t31-kappa_2.*t3.*t5.*t10.*t15.*t22.*t25.*t30-L.*kappa_1.*kappa_2.*t3.*t5.*t19.*t24.*t25.*w.*3.0-L.*kappa_2.*t3.*t5.*t15.*t19.*t23.*t31.*w.*2.0-L.*kappa_2.*t3.*t5.*t15.*t20.*t25.*t30.*w.*2.0-kappa_1.*kappa_2.*t2.*t5.*t15.*t17.*t20.*t24.*t31.*2.0-kappa_1.*kappa_2.*t2.*t5.*t15.*t19.*t21.*t24.*t30.*2.0-kappa_1.*kappa_2.*t2.*t5.*t15.*t21.*t24.*t30.*t34.*2.0-kappa_1.*kappa_2.*t2.*t5.*t15.*t21.*t24.*t31.*t34.*2.0-L.*kappa_1.*kappa_2.*t5.*t15.*t17.*t22.*t24.*t31.*w-L.*kappa_1.*kappa_2.*t5.*t15.*t19.*t23.*t24.*t31.*w-kappa_1.*kappa_2.*t3.*t5.*t10.*t15.*t17.*t22.*t24.*t31-kappa_1.*kappa_2.*t3.*t5.*t10.*t15.*t19.*t23.*t24.*t31-L.*kappa_1.*kappa_2.*t3.*t5.*t15.*t17.*t20.*t24.*t31.*w.*2.0-L.*kappa_1.*kappa_2.*t3.*t5.*t15.*t19.*t21.*t24.*t30.*w.*2.0-L.*kappa_1.*kappa_2.*t3.*t5.*t15.*t21.*t24.*t30.*t34.*w.*2.0-L.*kappa_1.*kappa_2.*t3.*t5.*t15.*t21.*t24.*t31.*t34.*w.*2.0)-t148.*t183.*(t35-t36+t37+t38-t39+t40+t41-t42+t43-t44+t45-t46+t47+t48-t49+t50+t51-t52+t53-t54+t87+t91+t95+t101+t106+t110+t114+t120+t207+t208+t209+t210+t211+t212+t213+t214+t215+t216+t217+t347+t348+t350+t351+t352+t354+t356+t358+t359+t360+t361+t362+t363+t364+t365+t366-kappa_2.*t2.*t5.*t19.*t25.*2.0-kappa_2.*t2.*t3.*t5.*t19.*t25.*2.0-kappa_2.*t3.*t5.*t10.*t17.*t34-L.*kappa_2.*t5.*t17.*t34.*w-L.*kappa_2.*t3.*t5.*t19.*t25.*w.*3.0-kappa_2.*t2.*t5.*t15.*t17.*t22.*t30.*2.0-kappa_2.*t2.*t5.*t15.*t17.*t22.*t31.*2.0-kappa_2.*t2.*t5.*t15.*t22.*t25.*t31.*2.0-L.*kappa_1.*kappa_2.*t5.*t17.*t19.*t24.*w-L.*kappa_1.*kappa_2.*t5.*t24.*t25.*t34.*w-L.*kappa_2.*t5.*t15.*t20.*t25.*t30.*w-kappa_1.*kappa_2.*t3.*t5.*t10.*t17.*t19.*t24-kappa_1.*kappa_2.*t3.*t5.*t10.*t24.*t25.*t34-kappa_2.*t3.*t5.*t10.*t15.*t20.*t25.*t30-L.*kappa_2.*t3.*t5.*t15.*t17.*t22.*t30.*w.*2.0-L.*kappa_2.*t3.*t5.*t15.*t17.*t22.*t31.*w.*2.0-L.*kappa_2.*t3.*t5.*t15.*t22.*t25.*t31.*w.*2.0-kappa_1.*kappa_2.*t2.*t5.*t15.*t17.*t22.*t24.*t30.*2.0-kappa_1.*kappa_2.*t2.*t5.*t15.*t19.*t21.*t24.*t30.*2.0-kappa_1.*kappa_2.*t2.*t5.*t15.*t22.*t24.*t25.*t30.*2.0-kappa_1.*kappa_2.*t2.*t5.*t15.*t22.*t24.*t25.*t31.*2.0-kappa_1.*kappa_2.*t2.*t5.*t15.*t21.*t24.*t31.*t34.*2.0-L.*kappa_1.*kappa_2.*t5.*t15.*t17.*t20.*t24.*t31.*w-kappa_1.*kappa_2.*t3.*t5.*t10.*t15.*t17.*t20.*t24.*t31-L.*kappa_1.*kappa_2.*t3.*t5.*t15.*t17.*t22.*t24.*t30.*w.*2.0-L.*kappa_1.*kappa_2.*t3.*t5.*t15.*t19.*t21.*t24.*t30.*w.*2.0-L.*kappa_1.*kappa_2.*t3.*t5.*t15.*t22.*t24.*t25.*t30.*w.*2.0-L.*kappa_1.*kappa_2.*t3.*t5.*t15.*t22.*t24.*t25.*t31.*w.*2.0-L.*kappa_1.*kappa_2.*t3.*t5.*t15.*t21.*t24.*t31.*t34.*w.*2.0))+t184.*t289.*thetap, ...
                         deltap_o.*(t184.*(t133+t135+t137+t141+t144+t146-t189-t190-R.*kappa_2.*t2.*t5.*t15.*t22.*t25.*2.0+L.*R.*kappa_2.*t5.*t15.*t20.*t25.*w+R.*kappa_2.*t3.*t5.*t10.*t15.*t20.*t25-L.*R.*kappa_2.*t3.*t5.*t15.*t22.*t25.*w.*2.0+R.*kappa_1.*kappa_2.*t2.*t5.*t15.*t17.*t22.*t24.*2.0-L.*R.*kappa_1.*kappa_2.*t5.*t15.*t17.*t20.*t24.*w-R.*kappa_1.*kappa_2.*t3.*t5.*t10.*t15.*t17.*t20.*t24+L.*R.*kappa_1.*kappa_2.*t3.*t5.*t15.*t17.*t22.*t24.*w.*2.0)+t183.*t635.*(t220+t221+t222+t223+t224+t225+t226+t227+t228+t229+t230+t231+t232+t233+t234-t290-t291-t292-t293-t294-t295-t296-t297-t298-t299-t300-t301-t302-t303-t304))-dalpha_2.*(t184.*(R.*kappa_2.*t2.*t15.*t19.*t23.*t122.*2.0-R.*kappa_2.*t2.*t15.*t20.*t25.*t122.*2.0+L.*R.*kappa_2.*t15.*t19.*t21.*t122.*w-L.*R.*kappa_2.*t15.*t22.*t25.*t122.*w+R.*kappa_2.*t3.*t10.*t15.*t19.*t21.*t122-R.*kappa_2.*t3.*t10.*t15.*t22.*t25.*t122+L.*R.*kappa_2.*t3.*t15.*t19.*t23.*t122.*w.*2.0-L.*R.*kappa_2.*t3.*t15.*t20.*t25.*t122.*w.*2.0+R.*kappa_1.*kappa_2.*t2.*t15.*t17.*t20.*t24.*t122.*2.0-R.*kappa_1.*kappa_2.*t2.*t15.*t19.*t21.*t24.*t122.*2.0+L.*R.*kappa_1.*kappa_2.*t15.*t17.*t22.*t24.*t122.*w+L.*R.*kappa_1.*kappa_2.*t15.*t19.*t23.*t24.*t122.*w+R.*kappa_1.*kappa_2.*t3.*t10.*t15.*t17.*t22.*t24.*t122+R.*kappa_1.*kappa_2.*t3.*t10.*t15.*t19.*t23.*t24.*t122+L.*R.*kappa_1.*kappa_2.*t3.*t15.*t17.*t20.*t24.*t122.*w.*2.0-L.*R.*kappa_1.*kappa_2.*t3.*t15.*t19.*t21.*t24.*t122.*w.*2.0)-t183.*t289.*t420)+deltap_i.*(t184.*(t124+t125+t129+t130+t132+t134+t136+t140+t142+t143+t145+t147-t185-t186-R.*t2.*t25.*t191.*2.0+R.*t10.*t25.*t191+R.*t2.*t15.*t21.*t31.*2.0-L.*R.*t15.*t23.*t31.*w+R.*kappa_1.*t2.*t17.*t24.*t191.*2.0-R.*kappa_1.*t10.*t17.*t24.*t191-R.*t3.*t10.*t15.*t23.*t31+R.*t10.*t15.*t21.*t31.*t191+R.*t2.*t23.*t31.*t198.*t199+L.*R.*t3.*t15.*t21.*t31.*w.*2.0+L.*R.*t15.*t23.*t31.*t191.*w.*2.0+L.*R.*t21.*t31.*t198.*t199.*w.*(1.0./2.0)-R.*kappa_2.*t2.*t5.*t15.*t19.*t21.*2.0+R.*kappa_1.*t2.*t15.*t23.*t24.*t31.*2.0+R.*t3.*t10.*t21.*t31.*t198.*t199.*(1.0./2.0)+R.*t2.*t15.*t23.*t30.*t203.*t205.*2.0+L.*R.*kappa_2.*t5.*t15.*t19.*t23.*w+L.*R.*kappa_1.*t15.*t21.*t24.*t31.*w+L.*R.*t3.*t23.*t31.*t198.*t199.*w+L.*R.*t15.*t21.*t30.*t203.*t205.*w+R.*kappa_2.*t3.*t5.*t10.*t15.*t19.*t23+R.*kappa_1.*t3.*t10.*t15.*t21.*t24.*t31-R.*kappa_2.*t5.*t10.*t15.*t19.*t21.*t191+R.*kappa_2.*t5.*t10.*t15.*t22.*t25.*t191+R.*kappa_1.*t10.*t15.*t23.*t24.*t31.*t191-R.*kappa_2.*t2.*t5.*t19.*t23.*t198.*t199+R.*kappa_2.*t2.*t5.*t20.*t25.*t198.*t199-R.*kappa_1.*t2.*t21.*t24.*t31.*t198.*t199+R.*t3.*t10.*t15.*t21.*t30.*t203.*t205-L.*R.*kappa_2.*t3.*t5.*t15.*t19.*t21.*w.*2.0+L.*R.*kappa_1.*t3.*t15.*t23.*t24.*t31.*w.*2.0-L.*R.*kappa_2.*t5.*t15.*t19.*t23.*t191.*w.*2.0+L.*R.*kappa_2.*t5.*t15.*t20.*t25.*t191.*w.*2.0-L.*R.*kappa_1.*t15.*t21.*t24.*t31.*t191.*w.*2.0-L.*R.*kappa_2.*t5.*t19.*t21.*t198.*t199.*w.*(1.0./2.0)+L.*R.*kappa_2.*t5.*t22.*t25.*t198.*t199.*w.*(1.0./2.0)+L.*R.*kappa_1.*t23.*t24.*t31.*t198.*t199.*w.*(1.0./2.0)+L.*R.*t3.*t15.*t23.*t30.*t203.*t205.*w.*2.0-R.*kappa_1.*kappa_2.*t2.*t5.*t15.*t19.*t23.*t24.*2.0-R.*kappa_2.*t3.*t5.*t10.*t19.*t21.*t198.*t199.*(1.0./2.0)+R.*kappa_2.*t3.*t5.*t10.*t22.*t25.*t198.*t199.*(1.0./2.0)+R.*kappa_1.*t3.*t10.*t23.*t24.*t31.*t198.*t199.*(1.0./2.0)-R.*kappa_1.*t2.*t15.*t21.*t24.*t30.*t203.*t205.*2.0-L.*R.*kappa_1.*kappa_2.*t5.*t15.*t19.*t21.*t24.*w-L.*R.*kappa_2.*t3.*t5.*t19.*t23.*t198.*t199.*w+L.*R.*kappa_2.*t3.*t5.*t20.*t25.*t198.*t199.*w-L.*R.*kappa_1.*t3.*t21.*t24.*t31.*t198.*t199.*w+L.*R.*kappa_1.*t15.*t23.*t24.*t30.*t203.*t205.*w-R.*kappa_1.*kappa_2.*t3.*t5.*t10.*t15.*t19.*t21.*t24-R.*kappa_1.*kappa_2.*t5.*t10.*t15.*t17.*t22.*t24.*t191-R.*kappa_1.*kappa_2.*t5.*t10.*t15.*t19.*t23.*t24.*t191-R.*kappa_1.*kappa_2.*t2.*t5.*t17.*t20.*t24.*t198.*t199+R.*kappa_1.*kappa_2.*t2.*t5.*t19.*t21.*t24.*t198.*t199+R.*kappa_1.*t3.*t10.*t15.*t23.*t24.*t30.*t203.*t205-L.*R.*kappa_1.*kappa_2.*t3.*t5.*t15.*t19.*t23.*t24.*w.*2.0-L.*R.*kappa_1.*kappa_2.*t5.*t15.*t17.*t20.*t24.*t191.*w.*2.0+L.*R.*kappa_1.*kappa_2.*t5.*t15.*t19.*t21.*t24.*t191.*w.*2.0-L.*R.*kappa_1.*kappa_2.*t5.*t17.*t22.*t24.*t198.*t199.*w.*(1.0./2.0)-L.*R.*kappa_1.*kappa_2.*t5.*t19.*t23.*t24.*t198.*t199.*w.*(1.0./2.0)-L.*R.*kappa_1.*t3.*t15.*t21.*t24.*t30.*t203.*t205.*w.*2.0-R.*kappa_1.*kappa_2.*t3.*t5.*t10.*t17.*t22.*t24.*t198.*t199.*(1.0./2.0)-R.*kappa_1.*kappa_2.*t3.*t5.*t10.*t19.*t23.*t24.*t198.*t199.*(1.0./2.0)-L.*R.*kappa_1.*kappa_2.*t3.*t5.*t17.*t20.*t24.*t198.*t199.*w+L.*R.*kappa_1.*kappa_2.*t3.*t5.*t19.*t21.*t24.*t198.*t199.*w)+t183.*t634.*(t220+t221+t222+t223+t224+t225+t226+t227+t228+t229+t230+t231+t232+t233+t234-t290-t291-t292-t293-t294-t295-t296-t297-t298-t299-t300-t301-t302-t303-t304))-dkappa_2.*(t184.*(R.*t2.*t5.*t15.*t19.*t23.*2.0-R.*t2.*t5.*t15.*t20.*t25.*2.0+L.*R.*t5.*t15.*t19.*t21.*w-L.*R.*t5.*t15.*t22.*t25.*w+R.*t3.*t5.*t10.*t15.*t19.*t21-R.*t3.*t5.*t10.*t15.*t22.*t25+L.*R.*t3.*t5.*t15.*t19.*t23.*w.*2.0-L.*R.*t3.*t5.*t15.*t20.*t25.*w.*2.0+R.*kappa_1.*t2.*t5.*t15.*t17.*t20.*t24.*2.0-R.*kappa_1.*t2.*t5.*t15.*t19.*t21.*t24.*2.0+L.*R.*kappa_1.*t5.*t15.*t17.*t22.*t24.*w+L.*R.*kappa_1.*t5.*t15.*t19.*t23.*t24.*w+R.*kappa_1.*t3.*t5.*t10.*t15.*t17.*t22.*t24+R.*kappa_1.*t3.*t5.*t10.*t15.*t19.*t23.*t24+L.*R.*kappa_1.*t3.*t5.*t15.*t17.*t20.*t24.*w.*2.0-L.*R.*kappa_1.*t3.*t5.*t15.*t19.*t21.*t24.*w.*2.0)-t183.*t288.*t289)-dkappa_1.*(t184.*(L.*R.*t17.*t24.*w-R.*t2.*t3.*t17.*t24.*2.0+R.*t3.*t10.*t17.*t24+R.*t2.*t15.*t21.*t24.*t31.*2.0-L.*R.*t15.*t23.*t24.*t31.*w-R.*t3.*t10.*t15.*t23.*t24.*t31+L.*R.*t3.*t15.*t21.*t24.*t31.*w.*2.0+R.*kappa_2.*t2.*t5.*t15.*t17.*t20.*t24.*2.0-R.*kappa_2.*t2.*t5.*t15.*t19.*t21.*t24.*2.0+L.*R.*kappa_2.*t5.*t15.*t17.*t22.*t24.*w+L.*R.*kappa_2.*t5.*t15.*t19.*t23.*t24.*w+R.*kappa_2.*t3.*t5.*t10.*t15.*t17.*t22.*t24+R.*kappa_2.*t3.*t5.*t10.*t15.*t19.*t23.*t24+L.*R.*kappa_2.*t3.*t5.*t15.*t17.*t20.*t24.*w.*2.0-L.*R.*kappa_2.*t3.*t5.*t15.*t19.*t21.*t24.*w.*2.0)-t183.*t289.*t457)-dalpha_1.*(t184.*(L.*R.*kappa_1.*t17.*t219.*w-R.*kappa_1.*t2.*t3.*t17.*t219.*2.0+R.*kappa_1.*t3.*t10.*t17.*t219+R.*kappa_1.*t2.*t15.*t21.*t31.*t219.*2.0-L.*R.*kappa_1.*t15.*t23.*t31.*t219.*w-R.*kappa_1.*t3.*t10.*t15.*t23.*t31.*t219+L.*R.*kappa_1.*t3.*t15.*t21.*t31.*t219.*w.*2.0+R.*kappa_1.*kappa_2.*t2.*t5.*t15.*t17.*t20.*t219.*2.0-R.*kappa_1.*kappa_2.*t2.*t5.*t15.*t19.*t21.*t219.*2.0+L.*R.*kappa_1.*kappa_2.*t5.*t15.*t17.*t22.*t219.*w+L.*R.*kappa_1.*kappa_2.*t5.*t15.*t19.*t23.*t219.*w+R.*kappa_1.*kappa_2.*t3.*t5.*t10.*t15.*t17.*t22.*t219+R.*kappa_1.*kappa_2.*t3.*t5.*t10.*t15.*t19.*t23.*t219+L.*R.*kappa_1.*kappa_2.*t3.*t5.*t15.*t17.*t20.*t219.*w.*2.0-L.*R.*kappa_1.*kappa_2.*t3.*t5.*t15.*t19.*t21.*t219.*w.*2.0)-t183.*t289.*t341)+t148.*t184.*thetap, ...
                         -deltap_o.*(R.*t7.*t15.*t184.*(t755+t756+t757-kappa_2.*t5.*t19.*t25).*2.0-R.*t7.*t15.*t183.*t635.*t640.*2.0)+dkappa_2.*(R.*t7.*t15.*t184.*(t5.*t17.*t19+t5.*t25.*t34+kappa_1.*t5.*t19.*t24.*t25-kappa_1.*t5.*t17.*t24.*t34).*2.0+R.*t7.*t15.*t183.*t288.*t640.*2.0)-dkappa_1.*(R.*t7.*t15.*t184.*(t17.*t24.*t30+t24.*t25.*t31-kappa_2.*t5.*t19.*t24.*t25+kappa_2.*t5.*t17.*t24.*t34).*2.0-R.*t7.*t15.*t183.*t457.*t640.*2.0)+deltap_i.*(R.*t7.*t15.*t184.*(t755+t756+t757+t17.*t30+t25.*t31-kappa_2.*t5.*t19.*t25-kappa_1.*t17.*t24.*t31+kappa_1.*t24.*t25.*t30-t17.*t30.*t203.*t205-t25.*t31.*t203.*t205+kappa_1.*t17.*t24.*t31.*t203.*t205-kappa_1.*t24.*t25.*t30.*t203.*t205).*2.0-R.*t7.*t184.*t198.*t199.*t640+R.*t7.*t15.*t183.*t634.*t640.*2.0-R.*t15.*t184.*t191.*t640.*w.*2.0)+dalpha_2.*(R.*t7.*t15.*t184.*(kappa_2.*t17.*t19.*t122+kappa_2.*t25.*t34.*t122+kappa_1.*kappa_2.*t19.*t24.*t25.*t122-kappa_1.*kappa_2.*t17.*t24.*t34.*t122).*2.0+R.*t7.*t15.*t183.*t420.*t640.*2.0)-dalpha_1.*(R.*t7.*t15.*t184.*(kappa_1.*t17.*t30.*t219+kappa_1.*t25.*t31.*t219-kappa_1.*kappa_2.*t5.*t19.*t25.*t219+kappa_1.*kappa_2.*t5.*t17.*t34.*t219).*2.0-R.*t7.*t15.*t183.*t341.*t640.*2.0), ...
                         0.0,0.0,dkappa_1.*(t24.*t184.*t932-t183.*t457.*t883.*t932)+dalpha_1.*(kappa_1.*t184.*t219.*t932-t183.*t341.*t883.*t932)+deltap_i.*(t184.*t883.*(t2.*t191.*t880.*-2.0-t2.*t191.*t881.*2.0+t10.*t191.*t880+t10.*t191.*t881+t10.*t15.*t17.*t21.*t30.*t191-t10.*t15.*t17.*t23.*t31.*t191+t10.*t15.*t21.*t25.*t31.*t191+t10.*t15.*t23.*t25.*t30.*t191+t2.*t17.*t21.*t31.*t198.*t199+t2.*t17.*t23.*t30.*t198.*t199-t2.*t21.*t25.*t30.*t198.*t199+t2.*t23.*t25.*t31.*t198.*t199+L.*t15.*t17.*t21.*t31.*t191.*w.*2.0+L.*t15.*t17.*t23.*t30.*t191.*w.*2.0-L.*t15.*t21.*t25.*t30.*t191.*w.*2.0+L.*t15.*t23.*t25.*t31.*t191.*w.*2.0+L.*t17.*t21.*t30.*t198.*t199.*w.*(1.0./2.0)-L.*t17.*t23.*t31.*t198.*t199.*w.*(1.0./2.0)+L.*t21.*t25.*t31.*t198.*t199.*w.*(1.0./2.0)+L.*t23.*t25.*t30.*t198.*t199.*w.*(1.0./2.0)+kappa_2.*t5.*t10.*t15.*t22.*t191.*t880+kappa_2.*t5.*t10.*t15.*t22.*t191.*t881+kappa_2.*t2.*t5.*t20.*t198.*t199.*t880+kappa_2.*t2.*t5.*t20.*t198.*t199.*t881+t3.*t10.*t17.*t21.*t30.*t198.*t199.*(1.0./2.0)-t3.*t10.*t17.*t23.*t31.*t198.*t199.*(1.0./2.0)+t3.*t10.*t21.*t25.*t31.*t198.*t199.*(1.0./2.0)+t3.*t10.*t23.*t25.*t30.*t198.*t199.*(1.0./2.0)+t2.*t15.*t17.*t21.*t30.*t203.*t205.*2.0-t2.*t15.*t17.*t23.*t31.*t203.*t205.*2.0+t2.*t15.*t21.*t25.*t31.*t203.*t205.*2.0+t2.*t15.*t23.*t25.*t30.*t203.*t205.*2.0+L.*kappa_2.*t5.*t15.*t20.*t191.*t880.*w.*2.0+L.*kappa_2.*t5.*t15.*t20.*t191.*t881.*w.*2.0+L.*kappa_2.*t5.*t22.*t198.*t199.*t880.*w.*(1.0./2.0)+L.*kappa_2.*t5.*t22.*t198.*t199.*t881.*w.*(1.0./2.0)+L.*t3.*t17.*t21.*t31.*t198.*t199.*w+L.*t3.*t17.*t23.*t30.*t198.*t199.*w-L.*t3.*t21.*t25.*t30.*t198.*t199.*w+L.*t3.*t23.*t25.*t31.*t198.*t199.*w-L.*t15.*t17.*t21.*t31.*t203.*t205.*w-L.*t15.*t17.*t23.*t30.*t203.*t205.*w+L.*t15.*t21.*t25.*t30.*t203.*t205.*w-L.*t15.*t23.*t25.*t31.*t203.*t205.*w+kappa_2.*t5.*t10.*t15.*t17.*t19.*t23.*t191-kappa_2.*t5.*t10.*t15.*t19.*t21.*t25.*t191+kappa_2.*t5.*t10.*t15.*t17.*t21.*t34.*t191+kappa_2.*t5.*t10.*t15.*t23.*t25.*t34.*t191-kappa_2.*t2.*t5.*t17.*t19.*t21.*t198.*t199-kappa_2.*t2.*t5.*t19.*t23.*t25.*t198.*t199+kappa_2.*t2.*t5.*t17.*t23.*t34.*t198.*t199-kappa_2.*t2.*t5.*t21.*t25.*t34.*t198.*t199+kappa_2.*t3.*t5.*t10.*t22.*t198.*t199.*t880.*(1.0./2.0)+kappa_2.*t3.*t5.*t10.*t22.*t198.*t199.*t881.*(1.0./2.0)-t3.*t10.*t15.*t17.*t21.*t31.*t203.*t205-t3.*t10.*t15.*t17.*t23.*t30.*t203.*t205+t3.*t10.*t15.*t21.*t25.*t30.*t203.*t205-t3.*t10.*t15.*t23.*t25.*t31.*t203.*t205-L.*kappa_2.*t5.*t15.*t17.*t19.*t21.*t191.*w.*2.0-L.*kappa_2.*t5.*t15.*t19.*t23.*t25.*t191.*w.*2.0+L.*kappa_2.*t5.*t15.*t17.*t23.*t34.*t191.*w.*2.0-L.*kappa_2.*t5.*t15.*t21.*t25.*t34.*t191.*w.*2.0+L.*kappa_2.*t5.*t17.*t19.*t23.*t198.*t199.*w.*(1.0./2.0)-L.*kappa_2.*t5.*t19.*t21.*t25.*t198.*t199.*w.*(1.0./2.0)+L.*kappa_2.*t5.*t17.*t21.*t34.*t198.*t199.*w.*(1.0./2.0)+L.*kappa_2.*t5.*t23.*t25.*t34.*t198.*t199.*w.*(1.0./2.0)+L.*kappa_2.*t3.*t5.*t20.*t198.*t199.*t880.*w+L.*kappa_2.*t3.*t5.*t20.*t198.*t199.*t881.*w+L.*t3.*t15.*t17.*t21.*t30.*t203.*t205.*w.*2.0-L.*t3.*t15.*t17.*t23.*t31.*t203.*t205.*w.*2.0+L.*t3.*t15.*t21.*t25.*t31.*t203.*t205.*w.*2.0+L.*t3.*t15.*t23.*t25.*t30.*t203.*t205.*w.*2.0+kappa_2.*t3.*t5.*t10.*t17.*t19.*t23.*t198.*t199.*(1.0./2.0)-kappa_2.*t3.*t5.*t10.*t19.*t21.*t25.*t198.*t199.*(1.0./2.0)+kappa_2.*t3.*t5.*t10.*t17.*t21.*t34.*t198.*t199.*(1.0./2.0)+kappa_2.*t3.*t5.*t10.*t23.*t25.*t34.*t198.*t199.*(1.0./2.0)-L.*kappa_2.*t3.*t5.*t17.*t19.*t21.*t198.*t199.*w-L.*kappa_2.*t3.*t5.*t19.*t23.*t25.*t198.*t199.*w+L.*kappa_2.*t3.*t5.*t17.*t23.*t34.*t198.*t199.*w-L.*kappa_2.*t3.*t5.*t21.*t25.*t34.*t198.*t199.*w)-t183.*t634.*t883.*t932)+dkappa_2.*(t184.*t883.*(t2.*t5.*t15.*t20.*t880.*2.0+t2.*t5.*t15.*t20.*t881.*2.0-t2.*t5.*t15.*t17.*t19.*t21.*2.0-t2.*t5.*t15.*t19.*t23.*t25.*2.0+t2.*t5.*t15.*t17.*t23.*t34.*2.0-t2.*t5.*t15.*t21.*t25.*t34.*2.0+t3.*t5.*t10.*t15.*t22.*t880+t3.*t5.*t10.*t15.*t22.*t881+L.*t5.*t15.*t22.*t880.*w+L.*t5.*t15.*t22.*t881.*w+L.*t5.*t15.*t17.*t19.*t23.*w-L.*t5.*t15.*t19.*t21.*t25.*w+L.*t5.*t15.*t17.*t21.*t34.*w+L.*t5.*t15.*t23.*t25.*t34.*w+L.*t3.*t5.*t15.*t20.*t880.*w.*2.0+L.*t3.*t5.*t15.*t20.*t881.*w.*2.0+t3.*t5.*t10.*t15.*t17.*t19.*t23-t3.*t5.*t10.*t15.*t19.*t21.*t25+t3.*t5.*t10.*t15.*t17.*t21.*t34+t3.*t5.*t10.*t15.*t23.*t25.*t34-L.*t3.*t5.*t15.*t17.*t19.*t21.*w.*2.0-L.*t3.*t5.*t15.*t19.*t23.*t25.*w.*2.0+L.*t3.*t5.*t15.*t17.*t23.*t34.*w.*2.0-L.*t3.*t5.*t15.*t21.*t25.*t34.*w.*2.0)-t183.*t288.*t883.*t932)+dalpha_2.*(t184.*t883.*(kappa_2.*t2.*t15.*t20.*t122.*t880.*2.0+kappa_2.*t2.*t15.*t20.*t122.*t881.*2.0+L.*kappa_2.*t15.*t22.*t122.*t880.*w+L.*kappa_2.*t15.*t22.*t122.*t881.*w-kappa_2.*t2.*t15.*t17.*t19.*t21.*t122.*2.0-kappa_2.*t2.*t15.*t19.*t23.*t25.*t122.*2.0+kappa_2.*t2.*t15.*t17.*t23.*t34.*t122.*2.0-kappa_2.*t2.*t15.*t21.*t25.*t34.*t122.*2.0+kappa_2.*t3.*t10.*t15.*t22.*t122.*t880+kappa_2.*t3.*t10.*t15.*t22.*t122.*t881+L.*kappa_2.*t15.*t17.*t19.*t23.*t122.*w-L.*kappa_2.*t15.*t19.*t21.*t25.*t122.*w+L.*kappa_2.*t15.*t17.*t21.*t34.*t122.*w+L.*kappa_2.*t15.*t23.*t25.*t34.*t122.*w+L.*kappa_2.*t3.*t15.*t20.*t122.*t880.*w.*2.0+L.*kappa_2.*t3.*t15.*t20.*t122.*t881.*w.*2.0+kappa_2.*t3.*t10.*t15.*t17.*t19.*t23.*t122-kappa_2.*t3.*t10.*t15.*t19.*t21.*t25.*t122+kappa_2.*t3.*t10.*t15.*t17.*t21.*t34.*t122+kappa_2.*t3.*t10.*t15.*t23.*t25.*t34.*t122-L.*kappa_2.*t3.*t15.*t17.*t19.*t21.*t122.*w.*2.0-L.*kappa_2.*t3.*t15.*t19.*t23.*t25.*t122.*w.*2.0+L.*kappa_2.*t3.*t15.*t17.*t23.*t34.*t122.*w.*2.0-L.*kappa_2.*t3.*t15.*t21.*t25.*t34.*t122.*w.*2.0)-t183.*t420.*t883.*t932)+deltap_o.*(t184.*t883.*(kappa_2.*t2.*t5.*t15.*t22.*t880.*-2.0-kappa_2.*t2.*t5.*t15.*t22.*t881.*2.0+L.*kappa_2.*t5.*t15.*t20.*t880.*w+L.*kappa_2.*t5.*t15.*t20.*t881.*w+kappa_2.*t2.*t5.*t15.*t17.*t19.*t23.*2.0-kappa_2.*t2.*t5.*t15.*t19.*t21.*t25.*2.0+kappa_2.*t2.*t5.*t15.*t17.*t21.*t34.*2.0+kappa_2.*t2.*t5.*t15.*t23.*t25.*t34.*2.0+kappa_2.*t3.*t5.*t10.*t15.*t20.*t880+kappa_2.*t3.*t5.*t10.*t15.*t20.*t881+L.*kappa_2.*t5.*t15.*t17.*t19.*t21.*w+L.*kappa_2.*t5.*t15.*t19.*t23.*t25.*w-L.*kappa_2.*t5.*t15.*t17.*t23.*t34.*w+L.*kappa_2.*t5.*t15.*t21.*t25.*t34.*w-L.*kappa_2.*t3.*t5.*t15.*t22.*t880.*w.*2.0-L.*kappa_2.*t3.*t5.*t15.*t22.*t881.*w.*2.0+kappa_2.*t3.*t5.*t10.*t15.*t17.*t19.*t21+kappa_2.*t3.*t5.*t10.*t15.*t19.*t23.*t25-kappa_2.*t3.*t5.*t10.*t15.*t17.*t23.*t34+kappa_2.*t3.*t5.*t10.*t15.*t21.*t25.*t34+L.*kappa_2.*t3.*t5.*t15.*t17.*t19.*t23.*w.*2.0-L.*kappa_2.*t3.*t5.*t15.*t19.*t21.*t25.*w.*2.0+L.*kappa_2.*t3.*t5.*t15.*t17.*t21.*t34.*w.*2.0+L.*kappa_2.*t3.*t5.*t15.*t23.*t25.*t34.*w.*2.0)-t183.*t635.*t883.*t932), ...
                         0.0,0.0,0.0,0.0,0.0,0.0,0.0,0.0,0.0,0.0,-L.*deltap_i.*t8.*t191.*w,0.0],[9,3]);
